simulink model "LDPC_sim"  (R2024a)
(part 11 of 20)

  LDPC Encoder : commblkcod2/LDPC Encoder  ParityCheckMat=sparse([55;2535;8598;9319;10220;14393;26910;27562;145;2625;8688;9409;10310;14483;27000;27652;235;2715;8778;9499;10400;14573;27090;27742;325;2805;8868;9589;10490;14663;27180;27832;415;2895;8958;9679;10580;14753;27270;27922;505;2985;9048;9769;10670;14843;27360;28012;595;3075;9138;9859;10760;14933;27450;28102;685;3165;9228;9949;10850;15023;27540;28192;775;3255;9318;10039;10940;15113;27630;28282;865;3345;9408;10129;11030;15203;27720;28372;955;3435;9498;10219;11120;15293;27810;28462;1045;3525;9588;10309;11210;15383;27900;28552;1135;3615;9678;10399;11300;15473;27990;28642;1225;3705;9768;10489;11390;15563;28080;28732;1315;3795;9858;10579;11480;15653;28170;28822;1405;3885;9948;10669;11570;15743;28260;28912;1495;3975;10038;10759;11660;15833;28350;29002;1585;4065;10128;10849;11750;15923;28440;29092;1675;4155;10218;10939;11840;16013;28530;29182;1765;4245;10308;11029;11930;16103;28620;29272;1855;4335;10398;11119;12020;16193;28710;29362;1945;4425;10488;11209;12110;16283;28800;29452;2035;4515;10578;11299;12200;16373;28890;29542;2125;4605;10668;11389;12290;16463;28980;29632;2215;4695;10758;11479;12380;16553;29070;29722;2305;4785;10848;11569;12470;16643;29160;29812;2395;4875;10938;11659;12560;16733;29250;29902;2485;4965;11028;11749;12650;16823;29340;29992;2575;5055;11118;11839;12740;16913;29430;30082;2665;5145;11208;11929;12830;17003;29520;30172;2755;5235;11298;12019;12920;17093;29610;30262;2845;5325;11388;12109;13010;17183;29700;30352;2935;5415;11478;12199;13100;17273;29790;30442;3025;5505;11568;12289;13190;17363;29880;30532;3115;5595;11658;12379;13280;17453;29970;30622;3205;5685;11748;12469;13370;17543;30060;30712;3295;5775;11838;12559;13460;17633;30150;30802;3385;5865;11928;12649;13550;17723;30240;30892;3475;5955;12018;12739;13640;17813;30330;30982;3565;6045;12108;12829;13730;17903;30420;31072;3655;6135;12198;12919;13820;17993;30510;31162;3745;6225;12288;13009;13910;18083;30600;31252;3835;6315;12378;13099;14000;18173;30690;31342;3925;6405;12468;13189;14090;18263;30780;31432;4015;6495;12558;13279;14180;18353;30870;31522;4105;6585;12648;13369;14270;18443;30960;31612;4195;6675;12738;13459;14360;18533;31050;31702;4285;6765;12828;13549;14450;18623;31140;31792;4375;6855;12918;13639;14540;18713;31230;31882;4465;6945;13008;13729;14630;18803;31320;31972;4555;7035;13098;13819;14720;18893;31410;32062;4645;7125;13188;13909;14810;18983;31500;32152;4735;7215;13278;13999;14900;19073;31590;32242;4825;7305;13368;14089;14990;19163;31680;32332;22;4915;7395;13458;14179;15080;19253;31770;112;5005;7485;13548;14269;15170;19343;31860;202;5095;7575;13638;14359;15260;19433;31950;292;5185;7665;13728;14449;15350;19523;32040;382;5275;7755;13818;14539;15440;19613;32130;472;5365;7845;13908;14629;15530;19703;32220;562;5455;7935;13998;14719;15620;19793;32310;652;5545;8025;14088;14809;15710;19883;32400;90;742;5635;8115;14178;14899;15800;19973;180;832;5725;8205;14268;14989;15890;20063;270;922;5815;8295;14358;15079;15980;20153;360;1012;5905;8385;14448;15169;16070;20243;450;1102;5995;8475;14538;15259;16160;20333;540;1192;6085;8565;14628;15349;16250;20423;630;1282;6175;8655;14718;15439;16340;20513;720;1372;6265;8745;14808;15529;16430;20603;810;1462;6355;8835;14898;15619;16520;20693;900;1552;6445;8925;14988;15709;16610;20783;990;1642;6535;9015;15078;15799;16700;20873;1080;1732;6625;9105;15168;15889;16790;20963;1170;1822;6715;9195;15258;15979;16880;21053;1260;1912;6805;9285;15348;16069;16970;21143;1350;2002;6895;9375;15438;16159;17060;21233;1440;2092;6985;9465;15528;16249;17150;21323;1530;2182;7075;9555;15618;16339;17240;21413;1620;2272;7165;9645;15708;16429;17330;21503;1710;2362;7255;9735;15798;16519;17420;21593;1800;2452;7345;9825;15888;16609;17510;21683;1890;2542;7435;9915;15978;16699;17600;21773;1980;2632;7525;10005;16068;16789;17690;21863;2070;2722;7615;10095;16158;16879;17780;21953;2160;2812;7705;10185;16248;16969;17870;22043;2250;2902;7795;10275;16338;17059;17960;22133;2340;2992;7885;10365;16428;17149;18050;22223;2430;3082;7975;10455;16518;17239;18140;22313;2520;3172;8065;10545 ...(+2551010 chars)true;true;true;true;true;true;true;true;true;true;true;true;true;true;true;true;true;true;true;true;true;true;true;true;true;true;true;true;true;true;true;true;true;true;true;true;true;true;true;true;true;true;true;true;true;true;true;true;true;true;true;true;true;true;true;true;true;true;true;true;true;true;true;true;true;true;true;true;true;true;true;true;true;true;true;true;true;true;true;true;true;true;true;true;true;true;true;true;true;true;true;true;true;true;true;true;true;true;true;true;true;true;true;true;true;true;true;true;true;true;true;true;true;true;true;true;true;true;true;true;true;true;true;true;true;true;true;true;true;true;true;true;true;true;true;true;true;true;true;true;true;true;true;true;true;true;true;true;true;true;true;true;true;true;true;true;true;true;true;true;true;true;true;true;true;true;true;true;true;true;true;true;true;true;true;true;true;true;true;true;true;true;true;true;true;true;true;true;true;true;true;true;true;true;true;true;true;true;true;true;true;true;true;true;true;true;true;true;true;true;true;true;true;true;true;true;true;true;true;true;true;true;true;true;true;true;true;true;true;true;true;true;true;true;true;true;true;true;true;true;true;true;true;true;true;true;true;true;true;true;true;true;true;true;true;true;true;true;true;true;true;true;true;true;true;true;true;true;true;true;true;true;true;true;true;true;true;true;true;true;true;true;true;true;true;true;true;true;true;true;true;true;true;true;true;true;true;true;true;true;true;true;true;true;true;true;true;true;true;true;true;true;true;true;true;true;true;true;true;true;true;true;true;true;true;true;true;true;true;true;true;true;true;true;true;true;true;true;true;true;true;true;true;true;true;true;true;true;true;true;true;true;true;true;true;true;true;true;true;true;true;true;true;true;true;true;true;true;true;true;true;true;true;true;true;true;true;true;true;true;true;true;true;true;true;true;true;true;true;true;true;true;true;true;true;true;true;true;true;true;true;true;true;true;true;true;true;true;true;true;true;true;true;true;true;true;true;true;true;true;true;true;true;true;true;true;true;true;true;true;true;true;true;true;true;true;true;true;true;true;true;true;true;true;true;true;true;true;true;true;true;true;true;true;true;true;true;true;true;true;true;true;true;true;true;true;true;true;true;true;true;true;true;true;true;true;true;true;true;true;true;true;true;true;true;true;true;true;true;true;true;true;true;true;true;true;true;true;true;true;true;true;true;true;true;true;true;true;true;true;true;true;true;true;true;true;true;true;true;true;true;true;true;true;true;true;true;true;true;true;true;true;true;true;true;true;true;true;true;true;true;true;true;true;true;true;true;true;true;true;true;true;true;true;true;true;true;true;true;true;true;true;true;true;true;true;true;true;true;true;true;true;true;true;true;true;true;true;true;true;true;true;true;true;true;true;true;true;true;true;true;true;true;true;true;true;true;true;true;true;true;true;true;true;true;true;true;true;true;true;true;true;true;true;true;true;true;true;true;true;true;true;true;true;true;true;true;true;true;true;true;true;true;true;true;true;true;true;true;true;true;true;true;true;true;true;true;true;true;true;true;true;true;true;true;true;true;true;true;true;true;true;true;true;true;true;true;true;true;true;true;true;true;true;true;true;true;true;true;true;true;true;true;true;true;true;true;true;true;true;true;true;true;true;true;true;true;true;true;true;true;true;true;true;true;true;true;true;true;true;true;true;true;true;true;true;true;true;true;true;true;true;true;true;true;true;true;true;true;true;true;true;true;true;true;true;true;true;true;true;true;true;true;true;true;true;true;true;true;true;true;true;true;true;true;true;true;true;true;true;true;true;true;true;true;true;true;true;true;true;true;true;true;true;true;true;true;true;true;true;true;true;true;true;true;true;true;true;true;true;true;true;true;true;true;true;true;true;true;true;true;true;true;true;true;true;true;true;true;true;true;true;true;true;true;true;true;true;true;true;true;true;true;true;true;true;true;true;true;true;true;true;true;true;true;true;true;true;true;true;true;true;true;true;true;true;true;true;true;true;true;true;true;true;true;true;true;true;true;true;true;true;true;true;true;true;true;true;true;true;true;true;true;true;true;true;true;true;true;true;true;true;true;true;true;true;true;true;true;true;true;true;true;true;true;true;true;true;true;true;true;true;true;true;true;true;true;true;true;true;true;true;true;true;true;true;true;true;true;true;true;true;true;true;true;true;true;true;true;true;true;true;true;true;true;true;true;true;true;true;true;true;true;true;true;true;true;true;true;true;true;true;true;true;true;true;true;true;true;true;true;true;true;true;true;true;true;true;true;true;true;true;true;true;true;true;true;true;true;true;true;true;true;true;true;true;true;true;true;true;true;true;true;true;true;true;true;true;true;true;true;true;true;true;true;true;true;true;true;true;true;true;true;true;true;true;true;true;true;true;true;true;true;true;true;true;true;true;true;true;true;true;true;true;true;true;true;true;true;true;true;true;true;true;true;true;true;true;true;true;true;true;true;true;true;true;true;true;true;true;true;true;true;true;true;true;true;true;true;true;true;true;true;true;true;true;true;true;true;true;true;true;true;true;true;true;true;true;true;true;true;true;true;true;true;true;true;true;true;true;true;true;true;true;true;true;true;true;true;true;true;true;true;true;true;true;true;true;true;true;true;true;true;true;true;true;true;true;true;true;true;true;true;true;true;true;true;true;true;true;true;true;true;true;true;true;true;true;true;true;true;true;true;true;true;true;true;true;true;true;true;true;true;true;true;true;true;true;true;true;true;true;true;true;true;true;true;true;true;true;true;true;true;true;true;true;true;true;true;true;true;true;true;true;true;true;true;true;true;true;true;true;true;true;true;true;true;true;true;true;true;true;true;true;true;true;true;true;true;true;true;true;true;true;true;true;true;true;true;true;true;true;true;true;true;true;true;true;true;true;true;true;true;true;true;true;true;true;true;true;true;true;true;true;true;true;true;true;true;true;true;true;true;true;true;true;true;true;true;true;true;true;true;true;true;true;true;true;true;true;true;true;true;true;true;true;true;true;true;true;true;true;true;true;true;true;true;true;true;true;true;true;true;true;true;true;true;true;true;true;true;true;true;true;true;true;true;true;true;true;true;true;true;true;true;true;true;true;true;true;true;true;true;true;true;true;true;true;true;true;true;true;true;true;true;true;true;true;true;true;true;true;true;true;true;true;true;true;true;true;true;true;true;true;true;true;true;true;true;true;true;true;true;true;true;true;true;true;true;true;true;true;true;true;true;true;true;true;true;true;true;true;true;true;true;true;true;true;true;true;true;true;true;true;true;true;true;true;true;true;true;true;true;true;true;true;true;true;true;true;true;true;true;true;true;true;true;true;true;true;true;true;true;true;true;true;true;true;true;true;true;true;true;true;true;true;true;true;true;true;true;true;true;true;true;true;true;true;true;true;true;true;true;true;true;true;true;true;true;true;true;true;true;true;true;true;true;true;true;true;true;true;true;true;true;true;true;true;true;true;true;true;true;true;true;true;true;true;true;true;true;true;true;true;true;true;true;true;true;true;true;true;true;true;true;true;true;true;true;true;true;true;true;true;true;true;true;true;true;true;true;true;true;true;true;true;true;true;true;true;true;true;true;true;true;true;true;true;true;true;true;true;true;true;true;true;true;true;true;true;true;true;true;true;true;true;true;true;true;true;true;true;true;true;true;true;true;true;true;true;true;true;true;true;true;true;true;true;true;true;true;true;true;true;true;true;true;true;true;true;true;true;true;true;true;true;true;true;true;true;true;true;true;true;true;true;true;true;true;true;true;true;true;true;true;true;true;true;true;true;true;true;true;true;true;true;true;true;true;true;true;true;true;true;true;true;true;true;true;true;true;true;true;true;true;true;true;true;true;true;true;true;true;true;true;true;true;true;true;true;true;true;true;true;true;true;true;true;true;true;true;true;true;true;true;true;true;true;true;true;true;true;true;true;true;true;true;true;true;true;true;true;true;true;true;true;true;true;true;true;true;true;true;true;true;true;true;true;true;true;true;true;true;true;true;true;true;true;true;true;true;true;true;true;true;true;true;true;true;true;true;true;true;true;true;true;true;true;true;true;true;true;true;true;true;true;true;true;true;true;true;true;true;true;true;true;true;true;true;true;true;true;true;true;true;true;true;true;true;true;true;true;true;true;true;true;true;true;true;true;true;true;true;true;true;true;true;true;true;true;true;true;true;true;true;true;true;true;true;true;true;true;true;true;true;true;true;true;true;true;true;true;true;true;true;true;true;true;true;true;true;true;true;true;true;true;true;true;true;true;true;true;true;true;true;true;true;true;true;true;true;true;true;true;true;true;true;true;true;true;true;true;true;true;true;true;true;true;true;true;true;true;true;true;true;true;true;true;true;true;true;true;true;true;true;true;true;true;true;true;true;true;true;true;true;true;true;true;true;true;true;true;true;true;true;true;true;true;true;true;true;true;true;true;true;true;true;true;true;true;true;true;true;true;true;true;true;true;true;true;true;true;true;true;true;true;true;true;true;true;true;true;true;true;true;true;true;true;true;true;true;true;true;true;true;true;true;true;true;true;true;true;true;true;true;true;true;true;true;true;true;true;true;true;true;true;true;true;true;true;true;true;true;true;true;true;true;true;true;true;true;true;true;true;true;true;true;true;true;true;true;true;true;true;true;true;true;true;true;true;true;true;true;true;true;true;true;true;true;true;true;true;true;true;true;true;true;true;true;true;true;true;true;true;true;true;true;true;true;true;true;true;true;true;true;true;true;true;true;true;true;true;true;true;true;true;true;true;true;true;true;true;true;true;true;true;true;true;true;true;true;true;true;true;true;true;true;true;true;true;true;true;true;true;true;true;true;true;true;true;true;true;true;true;true;true;true;true;true;true;true;true;true;true;true;true;true;true;true;true;true;true;true;true;true;true;true;true;true;true;true;true;true;true;true;true;true;true;true;true;true;true;true;true;true;true;true;true;true;true;true;true;true;true;true;true;true;true;true;true;true;true;true;true;true;true;true;true;true;true;true;true;true;true;true;true;true;true;true;true;true;true;true;true;true;true;true;true;true;true;true;true;true;true;true;true;true;true;true;true;true;true;true;true;true;true;true;true;true;true;true;true;true;true;true;true;true;true;true;true;true;true;true;true;true;true;true;true;true;true;true;true;true;true;true;true;true;true;true;true;true;true;true;true;true;true;true;true;true;true;true;true;true;true;true;true;true;true;true;true;true;true;true;true;true;true;true;true;true;true;true;true;true;true;true;true;true;true;true;true;true;true;true;true;true;true;true;true;true;true;true;true;true;true;true;true;true;true;true;true;true;true;true;true;true;true;true;true;true;true;true;true;true;true;true;true;true;true;true;true;true;true;true;true;true;true;true;true;true;true;true;true;true;true;true;true;true;true;true;true;true;true;true;true;true;true;true;true;true;true;true;true;true;true;true;true;true;true;true;true;true;true;true;true;true;true;true;true;true;true;true;true;true;true;true;true;true;true;true;true;true;true;true;true;true;true;true;true;true;true;true;true;true;true;true;true;true;true;true;true;true;true;true;true;true;true;true;true;true;true;true;true;true;true;true;true;true;true;true;true;true;true;true;true;true;true;true;true;true;true;true;true;true;true;true;true;true;true;true;true;true;true;true;true;true;true;true;true;true;true;true;true;true;true;true;true;true;true;true;true;true;true;true;true;true;true;true;true;true;true;true;true;true;true;true;true;true;true;true;true;true;true;true;true;true;true;true;true;true;true;true;true;true;true;true;true;true;true;true;true;true;true;true;true;true;true;true;true;true;true;true;true;true;true;true;true;true;true;true;true;true;true;true;true;true;true;true;true;true;true;true;true;true;true;true;true;true;true;true;true;true;true;true;true;true;true;true;true;true;true;true;true;true;true;true;true;true;true;true;true;true;true;true;true;true;true;true;true;true;true;true;true;true;true;true;true;true;true;true;true;true;true;true;true;true;true;true;true;true;true;true;true;true;true;true;true;true;true;true;true;true;true;true;true;true;true;true;true;true;true;true;true;true;true;true;true;true;true;true;true;true;true;true;true;true;true;true;true;true;true;true;true;true;true;true;true;true;true;true;true;true;true;true;true;true;true;true;true;true;true;true;true;true;true;true;true;true;true;true;true;true;true;true;true;true;true;true;true;true;true;true;true;true;true;true;true;true;true;true;true;true;true;true;true;true;true;true;true;true;true;true;true;true;true;true;true;true;true;true;true;true;true;true;true;true;true;true;true;true;true;true;true;true;true;true;true;true;true;true;true;true;true;true;true;true;true;true;true;true;true;true;true;true;true;true;true;true;true;true;true;true;true;true;true;true;true;true;true;true;true;true;true;true;true;true;true;true;true;true;true;true;true;true;true;true;true;true;true;true;true;true;true;true;true;true;true;true;true;true;true;true;true;true;true;true;true;true;true;true;true;true;true;true;true;true;true;true;true;true;true;true;true;true;true;true;true;true;true;true;true;true;true;true;true;true;true;true;true;true;true;true;true;true;true;true;true;true;true;true;true;true;true;true;true;true;true;true;true;true;true;true;true;true;true;true;true;true;true;true;true;true;true;true;true;true;true;true;true;true;true;true;true;true;true;true;true;true;true;true;true;true;true;true;true;true;true;true;true;true;true;true;true;true;true;true;true;true;true;true;true;true;true;true;true;true;true;true;true;true;true;true;true;true;true;true;true;true;true;true;true;true;true;true;true;true;true;true;true;true;true;true;true;true;true;true;true;true;true;true;true;true;true;true;true;true;true;true;true;true;true;true;true;true;true;true;true;true;true;true;true;true;true;true;true;true;true;true;true;true;true;true;true;true;true;true;true;true;true;true;true;true;true;true;true;true;true;true;true;true;true;true;true;true;true;true;true;true;true;true;true;true;true;true;true;true;true;true;true;true;true;true;true;true;true;true;true;true;true;true;true;true;true;true;true;true;true;true;true;true;true;true;true;true;true;true;true;true;true;true;true;true;true;true;true;true;true;true;true;true;true;true;true;true;true;true;true;true;true;true;true;true;true;true;true;true;true;true;true;true;true;true;true;true;true;true;true;true;true;true;true;true;true;true;true;true;true;true;true;true;true;true;true;true;true;true;true;true;true;true;true;true;true;true;true;true;true;true;true;true;true;true;true;true;true;true;true;true;true;true;true;true;true;true;true;true;true;true;true;true;true;true;true;true;true;true;true;true;true;true;true;true;true;true;true;true;true;true;true;true;true;true;true;true;true;true;true;true;true;true;true;true;true;true;true;true;true;true;true;true;true;true;true;true;true;true;true;true;true;true;true;true;true;true;true;true;true;true;true;true;true;true;true;true;true;true;true;true;true;true;true;true;true;true;true;true;true;true;true;true;true;true;true;true;true;true;true;true;true;true;true;true;true;true;true;true;true;true;true;true;true;true;true;true;true;true;true;true;true;true;true;true;true;true;true;true;true;true;true;true;true;true;true;true;true;true;true;true;true;true;true;true;true;true;true;true;true;true;true;true;true;true;true;true;true;true;true;true;true;true;true;true;true;true;true;true;true;true;true;true;true;true;true;true;true;true;true;true;true;true;true;true;true;true;true;true;true;true;true;true;true;true;true;true;true;true;true;true;true;true;true;true;true;true;true;true;true;true;true;true;true;true;true;true;true;true;true;true;true;true;true;true;true;true;true;true;true;true;true;true;true;true;true;true;true;true;true;true;true;true;true;true;true;true;true;true;true;true;true;true;true;true;true;true;true;true;true;true;true;true;true;true;true;true;true;true;true;true;true;true;true;true;true;true;true;true;true;true;true;true;true;true;true;true;true;true;true;true;true;true;true;true;true;true;true;true;true;true;true;true;true;true;true;true;true;true;true;true;true;true;true;true;true;true;true;true;true;true;true;true;true;true;true;true;true;true;true;true;true;true;true;true;true;true;true;true;true;true;true;true;true;true;true;true;true;true;true;true;true;true;true;true;true;true;true;true;true;true;true;true;true;true;true;true;true;true;true;true;true;true;true;true;true;true;true;true;true;true;true;true;true;true;true;true;true;true;true;true;true;true;true;true;true;true;true;true;true;true;true;true;true;true;true;true;true;true;true;true;true;true;true;true;true;true;true;true;true;true;true;true;true;true;true;true;true;true;true;true;true;true;true;true;true;true;true;true;true;true;true;true;true;true;true;true;true;true;true;true;true;true;true;true;true;true;true;true;true;true;true;true;true;true;true;true;true;true;true;true;true;true;true;true;true;true;true;true;true;true;true;true;true;true;true;true;true;true;true;true;true;true;true;true;true;true;true;true;true;true;true;true;true;true;true;true;true;true;true;true;true;true;true;true;true;true;true;true;true;true;true;true;true;true;true;true;true;true;true;true;true;true;true;true;true;true;true;true;true;true;true;true;true;true;true;true;true;true;true;true;true;true;true;true;true;true;true;true;true;true;true;true;true;true;true;true;true;true;true;true;true;true;true;true;true;true;true;true;true;true;true;true;true;true;true;true;true;true;true;true;true;true;true;true;true;true;true;true;true;true;true;true;true;true;true;true;true;true;true;true;true;true;true;true;true;true;true;true;true;true;true;true;true;true;true;true;true;true;true;true;true;true;true;true;true;true;true;true;true;true;true;true;true;true;true;true;true;true;true;true;true;true;true;true;true;true;true;true;true;true;true;true;true;true;true;true;true;true;true;true;true;true;true;true;true;true;true;true;true;true;true;true;true;true;true;true;true;true;true;true;true;true;true;true;true;true;true;true;true;true;true;true;true;true;true;true;true;true;true;true;true;true;true;true;true;true;true;true;true;true;true;true;true;true;true;true;true;true;true;true;true;true;true;true;true;true;true;true;true;true;true;true;true;true;true;true;true;true;true;true;true;true;true;true;true;true;true;true;true;true;true;true;true;true;true;true;true;true;true;true;true;true;true;true;true;true;true;true;true;true;true;true;true;true;true;true;true;true;true;true;true;true;true;true;true;true;true;true;true;true;true;true;true;true;true;true;true;true;true;true;true;true;true;true;true;true;true;true;true;true;true;true;true;true;true;true;true;true;true;true;true;true;true;true;true;true;true;true;true;true;true;true;true;true;true;true;true;true;true;true;true;true;true;true;true;true;true;true;true;true;true;true;true;true;true;true;true;true;true;true;true;true;true;true;true;true;true;true;true;true;true;true;true;true;true;true;true;true;true;true;true;true;true;true;true;true;true;true;true;true;true;true;true;true;true;true;true;true;true;true;true;true;true;true;true;true;true;true;true;true;true;true;true;true;true;true;true;true;true;true;true;true;true;true;true;true;true;true;true;true;true;true;true;true;true;true;true;true;true;true;true;true;true;true;true;true;true;true;true;true;true;true;true;true;true;true;true;true;true;true;true;true;true;true;true;true;true;true;true;true;true;true;true;true;true;true;true;true;true;true;true;true;true;true;true;true;true;true;true;true;true;true;true;true;true;true;true;true;true;true;true;true;true;true;true;true;true;true;true;true;true;true;true;true;true;true;true;true;true;true;true;true;true;true;true;true;true;true;true;true;true;true;true;true;true;true;true;true;true;true;true;true;true;true;true;true;true;true;true;true;true;true;true;true;true;true;true;true;true;true;true;true;true;true;true;true;true;true;true;true;true;true;true;true;true;true;true;true;true;true;true;true;true;true;true;true;true;true;true;true;true;true;true;true;true;true;true;true;true;true;true;true;true;true;true;true;true;true;true;true;true;true;true;true;true;true;true;true;true;true;true;true;true;true;true;true;true;true;true;true;true;true;true;true;true;true;true;true;true;true;true;true;true;true;true;true;true;true;true;true;true;true;true;true;true;true;true;true;true;true;true;true;true;true;true;true;true;true;true;true;true;true;true;true;true;true;true;true;true;true;true;true;true;true;true;true;true;true;true;true;true;true;true;true;true;true;true;true;true;true;true;true;true;true;true;true;true;true;true;true;true;true;true;true;true;true;true;true;true;true;true;true;true;true;true;true;true;true;true;true;true;true;true;true;true;true;true;true;true;true;true;true;true;true;true;true;true;true;true;true;true;true;true;true;true;true;true;true;true;true;true;true;true;true;true;true;true;true;true;true;true;true;true;true;true;true;true;true;true;true;true;true;true;true;true;true;true;true;true;true;true;true;true;true;true;true;true;true;true;true;true;true;true;true;true;true;true;true;true;true;true;true;true;true;true;true;true;true;true;true;true;true;true;true;true;true;true;true;true;true;true;true;true;true;true;true;true;true;true;true;true;true;true;true;true;true;true;true;true;true;true;true;true;true;true;true;true;true;true;true;true;true;true;true;true;true;true;true;true;true;true;true;true;true;true;true;true;true;true;true;true;true;true;true;true;true;true;true;true;true;true;true;true;true;true;true;true;true;true;true;true;true;true;true;true;true;true;true;true;true;true;true;true;true;true;true;true;true;true;true;true;true;true;true;true;true;true;true;true;true;true;true;true;true;true;true;true;true;true;true;true;true;true;true;true;true;true;true;true;true;true;true;true;true;true;true;true;true;true;true;true;true;true;true;true;true;true;true;true;true;true;true;true;true;true;true;true;true;true;true;true;true;true;true;true;true;true;true;true;true;true;true;true;true;true;true;true;true;true;true;true;true;true;true;true;true;true;true;true;true;true;true;true;true;true;true;true;true;true;true;true;true;true;true;true;true;true;true;true;true;true;true;true;true;true;true;true;true;true;true;true;true;true;true;true;true;true;true;true;true;true;true;true;true;true;true;true;true;true;true;true;true;true;true;true;true;true;true;true;true;true;true;true;true;true;true;true;true;true;true;true;true;true;true;true;true;true;true;true;true;true;true;true;true;true;true;true;true;true;true;true;true;true;true;true;true;true;true;true;true;true;true;true;true;true;true;true;true;true;true;true;true;true;true;true;true;true;true;true;true;true;true;true;true;true;true;true;true;true;true;true;true;true;true;true;true;true;true;true;true;true;true;true;true;true;true;true;true;true;true;true;true;true;true;true;true;true;true;true;true;true;true;true;true;true;true;true;true;true;true;true;true;true;true;true;true;true;true;true;true;true;true;true;true;true;true;true;true;true;true;true;true;true;true;true;true;true;true;true;true;true;true;true;true;true;true;true;true;true;true;true;true;true;true;true;true;true;true;true;true;true;true;true;true;true;true;true;true;true;true;true;true;true;true;true;true;true;true;true;true;true;true;true;true;true;true;true;true;true;true;true;true;true;true;true;true;true;true;true;true;true;true;true;true;true;true;true;true;true;true;true;true;true;true;true;true;true;true;true;true;true;true;true;true;true;true;true;true;true;true;true;true;true;true;true;true;true;true;true;true;true;true;true;true;true;true;true;true;true;true;true;true;true;true;true;true;true;true;true;true;true;true;true;true;true;true;true;true;true;true;true;true;true;true;true;true;true;true;true;true;true;true;true;true;true;true;true;true;true;true;true;true;true;true;true;true;true;true;true;true;true;true;true;true;true;true;true;true;true;true;true;true;true;true;true;true;true;true;true;true;true;true;true;true;true;true;true;true;true;true;true;true;true;true;true;true;true;true;true;true;true;true;true;true;true;true;true;true;true;true;true;true;true;true;true;true;true;true;true;true;true;true;true;true;true;true;true;true;true;true;true;true;true;true;true;true;true;true;true;true;true;true;true;true;true;true;true;true;true;true;true;true;true;true;true;true;true;true;true;true;true;true;true;true;true;true;true;true;true;true;true;true;true;true;true;true;true;true;true;true;true;true;true;true;true;true;true;true;true;true;true;true;true;true;true;true;true;true;true;true;true;true;true;true;true;true;true;true;true;true;true;true;true;true;true;true;true;true;true;true;true;true;true;true;true;true;true;true;true;true;true;true;true;true;true;true;true;true;true;true;true;true;true;true;true;true;true;true;true;true;true;true;true;true;true;true;true;true;true;true;true;true;true;true;true;true;true;true;true;true;true;true;true;true;true;true;true;true;true;true;true;true;true;true;true;true;true;true;true;true;true;true;true;true;true;true;true;true;true;true;true;true;true;true;true;true;true;true;true;true;true;true;true;true;true;true;true;true;true;true;true;true;true;true;true;true;true;true;true;true;true;true;true;true;true;true;true;true;true;true;true;true;true;true;true;true;true;true;true;true;true;true;true;true;true;true;true;true;true;true;true;true;true;true;true;true;true;true;true;true;true;true;true;true;true;true;true;true;true;true;true;true;true;true;true;true;true;true;true;true;true;true;true;true;true;true;true;true;true;true;true;true;true;true;true;true;true;true;true;true;true;true;true;true;true;true;true;true;true;true;true;true;true;true;true;true;true;true;true;true;true;true;true;true;true;true;true;true;true;true;true;true;true;true;true;true;true;true;true;true;true;true;true;true;true;true;true;true;true;true;true;true;true;true;true;true;true;true;true;true;true;true;true;true;true;true;true;true;true;true;true;true;true;true;true;true;true;true;true;true;true;true;true;true;true;true;true;true;true;true;true;true;true;true;true;true;true;true;true;true;true;true;true;true;true;true;true;true;true;true;true;true;true;true;true;true;true;true;true;true;true;true;true;true;true;true;true;true;true;true;true;true;true;true;true;true;true;true;true;true;true;true;true;true;true;true;true;true;true;true;true;true;true;true;true;true;true;true;true;true;true;true;true;true;true;true;true;true;true;true;true;true;true;true;true;true;true;true;true;true;true;true;true;true;true;true;true;true;true;true;true;true;true;true;true;true;true;true;true;true;true;true;true;true;true;true;true;true;true;true;true;true;true;true;true;true;true;true;true;true;true;true;true;true;true;true;true;true;true;true;true;true;true;true;true;true;true;true;true;true;true;true;true;true;true;true;true;true;true;true;true;true;true;true;true;true;true;true;true;true;true;true;true;true;true;true;true;true;true;true;true;true;true;true;true;true;true;true;true;true;true;true;true;true;true;true;true;true;true;true;true;true;true;true;true;true;true;true;true;true;true;true;true;true;true;true;true;true;true;true;true;true;true;true;true;true;true;true;true;true;true;true;true;true;true;true;true;true;true;true;true;true;true;true;true;true;true;true;true;true;true;true;true;true;true;true;true;true;true;true;true;true;true;true;true;true;true;true;true;true;true;true;true;true;true;true;true;true;true;true;true;true;true;true;true;true;true;true;true;true;true;true;true;true;true;true;true;true;true;true;true;true;true;true;true;true;true;true;true;true;true;true;true;true;true;true;true;true;true;true;true;true;true;true;true;true;true;true;true;true;true;true;true;true;true;true;true;true;true;true;true;true;true;true;true;true;true;true;true;true;true;true;true;true;true;true;true;true;true;true;true;true;true;true;true;true;true;true;true;true;true;true;true;true;true;true;true;true;true;true;true;true;true;true;true;true;true;true;true;true;true;true;true;true;true;true;true;true;true;true;true;true;true;true;true;true;true;true;true;true;true;true;true;true;true;true;true;true;true;true;true;true;true;true;true;true;true;true;true;true;true;true;true;true;true;true;true;true;true;true;true;true;true;true;true;true;true;true;true;true;true;true;true;true;true;true;true;true;true;true;true;true;true;true;true;true;true;true;true;true;true;true;true;true;true;true;true;true;true;true;true;true;true;true;true;true;true;true;true;true;true;true;true;true;true;true;true;true;true;true;true;true;true;true;true;true;true;true;true;true;true;true;true;true;true;true;true;true;true;true;true;true;true;true;true;true;true;true;true;true;true;true;true;true;true;true;true;true;true;true;true;true;true;true;true;true;true;true;true;true;true;true;true;true;true;true;true;true;true;true;true;true;true;true;true;true;true;true;true;true;true;true;true;true;true;true;true;true;true;true;true;true;true;true;true;true;true;true;true;true;true;true;true;true;true;true;true;true;true;true;true;true;true;true;true;true;true;true;true;true;true;true;true;true;true;true;true;true;true;true;true;true;true;true;true;true;true;true;true;true;true;true;true;true;true;true;true;true;true;true;true;true;true;true;true;true;true;true;true;true;true;true;true;true;true;true;true;true;true;true;true;true;true;true;true;true;true;true;true;true;true;true;true;true;true;true;true;true;true;true;true;true;true;true;true;true;true;true;true;true;true;true;true;true;true;true;true;true;true;true;true;true;true;true;true;true;true;true;true;true;true;true;true;true;true;true;true;true;true;true;true;true;true;true;true;true;true;true;true;true;true;true;true;true;true;true;true;true;true;true;true;true;true;true;true;true;true;true;true;true;true;true;true;true;true;true;true;true;true;true;true;true;true;true;true;true;true;true;true;true;true;true;true;true;true;true;true;true;true;true;true;true;true;true;true;true;true;true;true;true;true;true;true;true;true;true;true;true;true;true;true;true;true;true;true;true;true;true;true;true;true;true;true;true;true;true;true;true;true;true;true;true;true;true;true;true;true;true;true;true;true;true;true;true;true;true;true;true;true;true;true;true;true;true;true;true;true;true;true;true;true;true;true;true;true;true;true;true;true;true;true;true;true;true;true;true;true;true;true;true;true;true;true;true;true;true;true;true;true;true;true;true;true;true;true;true;true;true;true;true;true;true;true;true;true;true;true;true;true;true;true;true;true;true;true;true;true;true;true;true;true;true;true;true;true;true;true;true;true;true;true;true;true;true;true;true;true;true;true;true;true;true;true;true;true;true;true;true;true;true;true;true;true;true;true;true;true;true;true;true;true;true;true;true;true;true;true;true;true;true;true;true;true;true;true;true;true;true;true;true;true;true;true;true;true;true;true;true;true;true;true;true;true;true;true;true;true;true;true;true;true;true;true;true;true;true;true;true;true;true;true;true;true;true;true;true;true;true;true;true;true;true;true;true;true;true;true;true;true;true;true;true;true;true;true;true;true;true;true;true;true;true;true;true;true;true;true;true;true;true;true;true;true;true;true;true;true;true;true;true;true;true;true;true;true;true;true;true;true;true;true;true;true;true;true;true;true;true;true;true;true;true;true;true;true;true;true;true;true;true;true;true;true;true;true;true;true;true;true;true;true;true;true;true;true;true;true;true;true;true;true;true;true;true;true;true;true;true;true;true;true;true;true;true;true;true;true;true;true;true;true;true;true;true;true;true;true;true;true;true;true;true;true;true;true;true;true;true;true;true;true;true;true;true;true;true;true;true;true;true;true;true;true;true;true;true;true;true;true;true;true;true;true;true;true;true;true;true;true;true;true;true;true;true;true;true;true;true;true;true;true;true;true;true;true;true;true;true;true;true;true;true;true;true;true;true;true;true;true;true;true;true;true;true;true;true;true;true;true;true;true;true;true;true;true;true;true;true;true;true;true;true;true;true;true;true;true;true;true;true;true;true;true;true;true;true;true;true;true;true;true;true;true;true;true;true;true;true;true;true;true;true;true;true;true;true;true;true;true;true;true;true;true;true;true;true;true;true;true;true;true;true;true;true;true;true;true;true;true;true;true;true;true;true;true;true;true;true;true;true;true;true;true;true;true;true;true;true;true;true;true;true;true;true;true;true;true;true;true;true;true;true;true;true;true;true;true;true;true;true;true;true;true;true;true;true;true;true;true;true;true;true;true;true;true;true;true;true;true;true;true;true;true;true;true;true;true;true;true;true;true;true;true;true;true;true;true;true;true;true;true;true;true;true;true;true;true;true;true;true;true;true;true;true;true;true;true;true;true;true;true;true;true;true;true;true;true;true;true;true;true;true;true;true;true;true;true;true;true;true;true;true;true;true;true;true;true;true;true;true;true;true;true;true;true;true;true;true;true;true;true;true;true;true;true;true;true;true;true;true;true;true;true;true;true;true;true;true;true;true;true;true;true;true;true;true;true;true;true;true;true;true;true;true;true;true;true;true;true;true;true;true;true;true;true;true;true;true;true;true;true;true;true;true;true;true;true;true;true;true;true;true;true;true;true;true;true;true;true;true;true;true;true;true;true;true;true;true;true;true;true;true;true;true;true;true;true;true;true;true;true;true;true;true;true;true;true;true;true;true;true;true;true;true;true;true;true;true;true;true;true;true;true;true;true;true;true;true;true;true;true;true;true;true;true;true;true;true;true;true;true;true;true;true;true;true;true;true;true;true;true;true;true;true;true;true;true;true;true;true;true;true;true;true;true;true;true;true;true;true;true;true;true;true;true;true;true;true;true;true;true;true;true;true;true;true;true;true;true;true;true;true;true;true;true;true;true;true;true;true;true;true;true;true;true;true;true;true;true;true;true;true;true;true;true;true;true;true;true;true;true;true;true;true;true;true;true;true;true;true;true;true;true;true;true;true;true;true;true;true;true;true;true;true;true;true;true;true;true;true;true;true;true;true;true;true;true;true;true;true;true;true;true;true;true;true;true;true;true;true;true;true;true;true;true;true;true;true;true;true;true;true;true;true;true;true;true;true;true;true;true;true;true;true;true;true;true;true;true;true;true;true;true;true;true;true;true;true;true;true;true;true;true;true;true;true;true;true;true;true;true;true;true;true;true;true;true;true;true;true;true;true;true;true;true;true;true;true;true;true;true;true;true;true;true;true;true;true;true;true;true;true;true;true;true;true;true;true;true;true;true;true;true;true;true;true;true;true;true;true;true;true;true;true;true;true;true;true;true;true;true;true;true;true;true;true;true;true;true;true;true;true;true;true;true;true;true;true;true;true;true;true;true;true;true;true;true;true;true;true;true;true;true;true;true;true;true;true;true;true;true;true;true;true;true;true;true;true;true;true;true;true;true;true;true;true;true;true;true;true;true;true;true;true;true;true;true;true;true;true;true;true;true;true;true;true;true;true;true;true;true;true;true;true;true;true;true;true;true;true;true;true;true;true;true;true;true;true;true;true;true;true;true;true;true;true;true;true;true;true;true;true;true;true;true;true;true;true;true;true;true;true;true;true;true;true;true;true;true;true;true;true;true;true;true;true;true;true;true;true;true;true;true;true;true;true;true;true;true;true;true;true;true;true;true;true;true;true;true;true;true;true;true;true;true;true;true;true;true;true;true;true;true;true;true;true;true;true;true;true;true;true;true;true;true;true;true;true;true;true;true;true;true;true;true;true;true;true;true;true;true;true;true;true;true;true;true;true;true;true;true;true;true;true;true;true;true;true;true;true;true;true;true;true;true;true;true;true;true;true;true;true;true;true;true;true;true;true;true;true;true;true;true;true;true;true;true;true;true;true;true;true;true;true;true;true;true;true;true;true;true;true;true;true;true;true;true;true;true;true;true;true;true;true;true;true;true;true;true;true;true;true;true;true;true;true;true;true;true;true;true;true;true;true;true;true;true;true;true;true;true;true;true;true;true;true;true;true;true;true;true;true;true;true;true;true;true;true;true;true;true;true;true;true;true;true;true;true;true;true;true;true;true;true;true;true;true;true;true;true;true;true;true;true;true;true;true;true;true;true;true;true;true;true;true;true;true;true;true;true;true;true;true;true;true;true;true;true;true;true;true;true;true;true;true;true;true;true;true;true;true;true;true;true;true;true;true;true;true;true;true;true;true;true;true;true;true;true;true;true;true;true;true;true;true;true;true;true;true;true;true;true;true;true;true;true;true;true;true;true;true;true;true;true;true;true;true;true;true;true;true;true;true;true;true;true;true;true;true;true;true;true;true;true;true;true;true;true;true;true;true;true;true;true;true;true;true;true;true;true;true;true;true;true;true;true;true;true;true;true;true;true;true;true;true;true;true;true;true;true;true;true;true;true;true;true;true;true;true;true;true;true;true;true;true;true;true;true;true;true;true;true;true;true;true;true;true;true;true;true;true;true;true;true;true;true;true;true;true;true;true;true;true;true;true;true;true;true;true;true;true;true;true;true;true;true;true;true;true;true;true;true;true;true;true;true;true;true;true;true;true;true;true;true;true;true;true;true;true;true;true;true;true;true;true;true;true;true;true;true;true;true;true;true;true;true;true;true;true;true;true;true;true;true;true;true;true;true;true;true;true;true;true;true;true;true;true;true;true;true;true;true;true;true;true;true;true;true;true;true;true;true;true;true;true;true;true;true;true;true;true;true;true;true;true;true;true;true;true;true;true;true;true;true;true;true;true;true;true;true;true;true;true;true;true;true;true;true;true;true;true;true;true;true;true;true;true;true;true;true;true;true;true;true;true;true;true;true;true;true;true;true;true;true;true;true;true;true;true;true;true;true;true;true;true;true;true;true;true;true;true;true;true;true;true;true;true;true;true;true;true;true;true;true;true;true;true;true;true;true;true;true;true;true;true;true;true;true;true;true;true;true;true;true;true;true;true;true;true;true;true;true;true;true;true;true;true;true;true;true;true;true;true;true;true;true;true;true;true;true;true;true;true;true;true;true;true;true;true;true;true;true;true;true;true;true;true;true;true;true;true;true;true;true;true;true;true;true;true;true;true;true;true;true;true;true;true;true;true;true;true;true;true;true;true;true;true;true;true;true;true;true;true;true;true;true;true;true;true;true;true;true;true;true;true;true;true;true;true;true;true;true;true;true;true;true;true;true;true;true;true;true;true;true;true;true;true;true;true;true;true;true;true;true;true;true;true;true;true;true;true;true;true;true;true;true;true;true;true;true;true;true;true;true;true;true;true;true;true;true;true;true;true;true;true;true;true;true;true;true;true;true;true;true;true;true;true;true;true;true;true;true;true;true;true;true;true;true;true;true;true;true;true;true;true;true;true;true;true;true;true;true;true;true;true;true;true;true;true;true;true;true;true;true;true;true;true;true;true;true;true;true;true;true;true;true;true;true;true;true;true;true;true;true;true;true;true;true;true;true;true;true;true;true;true;true;true;true;true;true;true;true;true;true;true;true;true;true;true;true;true;true;true;true;true;true;true;true;true;true;true;true;true;true;true;true;true;true;true;true;true;true;true;true;true;true;true;true;true;true;true;true;true;true;true;true;true;true;true;true;true;true;true;true;true;true;true;true;true;true;true;true;true;true;true;true;true;true;true;true;true;true;true;true;true;true;true;true;true;true;true;true;true;true;true;true;true;true;true;true;true;true;true;true;true;true;true;true;true;true;true;true;true;true;true;true;true;true;true;true;true;true;true;true;true;true;true;true;true;true;true;true;true;true;true;true;true;true;true;true;true;true;true;true;true;true;true;true;true;true;true;true;true;true;true;true;true;true;true;true;true;true;true;true;true;true;true;true;true;true;true;true;true;true;true;true;true;true;true;true;true;true;true;true;true;true;true;true;true;true;true;true;true;true;true;true;true;true;true;true;true;true;true;true;true;true;true;true;true;true;true;true;true;true;true;true;true;true;true;true;true;true;true;true;true;true;true;true;true;true;true;true;true;true;true;true;true;true;true;true;true;true;true;true;true;true;true;true;true;true;true;true;true;true;true;true;true;true;true;true;true;true;true;true;true;true;true;true;true;true;true;true;true;true;true;true;true;true;true;true;true;true;true;true;true;true;true;true;true;true;true;true;true;true;true;true;true;true;true;true;true;true;true;true;true;true;true;true;true;true;true;true;true;true;true;true;true;true;true;true;true;true;true;true;true;true;true;true;true;true;true;true;true;true;true;true;true;true;true;true;true;true;true;true;true;true;true;true;true;true;true;true;true;true;true;true;true;true;true;true;true;true;true;true;true;true;true;true;true;true;true;true;true;true;true;true;true;true;true;true;true;true;true;true;true;true;true;true;true;true;true;true;true;true;true;true;true;true;true;true;true;true;true;true;true;true;true;true;true;true;true;true;true;true;true;true;true;true;true;true;true;true;true;true;true;true;true;true;true;true;true;true;true;true;true;true;true;true;true;true;true;true;true;true;true;true;true;true;true;true;true;true;true;true;true;true;true;true;true;true;true;true;true;true;true;true;true;true;true;true;true;true;true;true;true;true;true;true;true;true;true;true;true;true;true;true;true;true;true;true;true;true;true;true;true;true;true;true;true;true;true;true;true;true;true;true;true;true;true;true;true;true;true;true;true;true;true;true;true;true;true;true;true;true;true;true;true;true;true;true;true;true;true;true;true;true;true;true;true;true;true;true;true;true;true;true;true;true;true;true;true;true;true;true;true;true;true;true;true;true;true;true;true;true;true;true;true;true;true;true;true;true;true;true;true;true;true;true;true;true;true;true;true;true;true;true;true;true;true;true;true;true;true;true;true;true;true;true;true;true;true;true;true;true;true;true;true;true;true;true;true;true;true;true;true;true;true;true;true;true;true;true;true;true;true;true;true;true;true;true;true;true;true;true;true;true;true;true;true;true;true;true;true;true;true;true;true;true;true;true;true;true;true;true;true;true;true;true;true;true;true;true;true;true;true;true;true;true;true;true;true;true;true;true;true;true;true;true;true;true;true;true;true;true;true;true;true;true;true;true;true;true;true;true;true;true;true;true;true;true;true;true;true;true;true;true;true;true;true;true;true;true;true;true;true;true;true;true;true;true;true;true;true;true;true;true;true;true;true;true;true;true;true;true;true;true;true;true;true;true;true;true;true;true;true;true;true;true;true;true;true;true;true;true;true;true;true;true;true;true;true;true;true;true;true;true;true;true;true;true;true;true;true;true;true;true;true;true;true;true;true;true;true;true;true;true;true;true;true;true;true;true;true;true;true;true;true;true;true;true;true;true;true;true;true;true;true;true;true;true;true;true;true;true;true;true;true;true;true;true;true;true;true;true;true;true;true;true;true;true;true;true;true;true;true;true;true;true;true;true;true;true;true;true;true;true;true;true;true;true;true;true;true;true;true;true;true;true;true;true;true;true;true;true;true;true;true;true;true;true;true;true;true;true;true;true;true;true;true;true;true;true;true;true;true;true;true;true;true;true;true;true;true;true;true;true;true;true;true;true;true;true;true;true;true;true;true;true;true;true;true;true;true;true;true;true;true;true;true;true;true;true;true;true;true;true;true;true;true;true;true;true;true;true;true;true;true;true;true;true;true;true;true;true;true;true;true;true;true;true;true;true;true;true;true;true;true;true;true;true;true;true;true;true;true;true;true;true;true;true;true;true;true;true;true;true;true;true;true;true;true;true;true;true;true;true;true;true;true;true;true;true;true;true;true;true;true;true;true;true;true;true;true;true;true;true;true;true;true;true;true;true;true;true;true;true;true;true;true;true;true;true;true;true;true;true;true;true;true;true;true;true;true;true;true;true;true;true;true;true;true;true;true;true;true;true;true;true;true;true;true;true;true;true;true;true;true;true;true;true;true;true;true;true;true;true;true;true;true;true;true;true;true;true;true;true;true;true;true;true;true;true;true;true;true;true;true;true;true;true;true;true;true;true;true;true;true;true;true;true;true;true;true;true;true;true;true;true;true;true;true;true;true;true;true;true;true;true;true;true;true;true;true;true;true;true;true;true;true;true;true;true;true;true;true;true;true;true;true;true;true;true;true;true;true;true;true;true;true;true;true;true;true;true;true;true;true;true;true;true;true;true;true;true;true;true;true;true;true;true;true;true;true;true;true;true;true;true;true;true;true;true;true;true;true;true;true;true;true;true;true;true;true;true;true;true;true;true;true;true;true;true;true;true;true;true;true;true;true;true;true;true;true;true;true;true;true;true;true;true;true;true;true;true;true;true;true;true;true;true;true;true;true;true;true;true;true;true;true;true;true;true;true;true;true;true;true;true;true;true;true;true;true;true;true;true;true;true;true;true;true;true;true;true;true;true;true;true;true;true;true;true;true;true;true;true;true;true;true;true;true;true;true;true;true;true;true;true;true;true;true;true;true;true;true;true;true;true;true;true;true;true;true;true;true;true;true;true;true;true;true;true;true;true;true;true;true;true;true;true;true;true;true;true;true;true;true;true;true;true;true;true;true;true;true;true;true;true;true;true;true;true;true;true;true;true;true;true;true;true;true;true;true;true;true;true;true;true;true;true;true;true;true;true;true;true;true;true;true;true;true;true;true;true;true;true;true;true;true;true;true;true;true;true;true;true;true;true;true;true;true;true;true;true;true;true;true;true;true;true;true;true;true;true;true;true;true;true;true;true;true;true;true;true;true;true;true;true;true;true;true;true;true;true;true;true;true;true;true;true;true;true;true;true;true;true;true;true;true;true;true;true;true;true;true;true;true;true;true;true;true;true;true;true;true;true;true;true;true;true;true;true;true;true;true;true;true;true;true;true;true;true;true;true;true;true;true;true;true;true;true;true;true;true;true;true;true;true;true;true;true;true;true;true;true;true;true;true;true;true;true;true;true;true;true;true;true;true;true;true;true;true;true;true;true;true;true;true;true;true;true;true;true;true;true;true;true;true;true;true;true;true;true;true;true;true;true;true;true;true;true;true;true;true;true;true;true;true;true;true;true;true;true;true;true;true;true;true;true;true;true;true;true;true;true;true;true;true;true;true;true;true;true;true;true;true;true;true;true;true;true;true;true;true;true;true;true;true;true;true;true;true;true;true;true;true;true;true;true;true;true;true;true;true;true;true;true;true;true;true;true;true;true;true;true;true;true;true;true;true;true;true;true;true;true;true;true;true;true;true;true;true;true;true;true;true;true;true;true;true;true;true;true;true;true;true;true;true;true;true;true;true;true;true;true;true;true;true;true;true;true;true;true;true;true;true;true;true;true;true;true;true;true;true;true;true;true;true;true;true;true;true;true;true;true;true;true;true;true;true;true;true;true;true;true;true;true;true;true;true;true;true;true;true;true;true;true;true;true;true;true;true;true;true;true;true;true;true;true;true;true;true;true;true;true;true;true;true;true;true;true;true;true;true;true;true;true;true;true;true;true;true;true;true;true;true;true;true;true;true;true;true;true;true;true;true;true;true;true;true;true;true;true;true;true;true;true;true;true;true;true;true;true;true;true;true;true;true;true;true;true;true;true;true;true;true;true;true;true;true;true;true;true;true;true;true;true;true;true;true;true;true;true;true;true;true;true;true;true;true;true;true;true;true;true;true;true;true;true;true;true;true;true;true;true;true;true;true;true;true;true;true;true;true;true;true;true;true;true;true;true;true;true;true;true;true;true;true;true;true;true;true;true;true;true;true;true;true;true;true;true;true;true;true;true;true;true;true;true;true;true;true;true;true;true;true;true;true;true;true;true;true;true;true;true;true;true;true;true;true;true;true;true;true;true;true;true;true;true;true;true;true;true;true;true;true;true;true;true;true;true;true;true;true;true;true;true;true;true;true;true;true;true;true;true;true;true;true;true;true;true;true;true;true;true;true;true;true;true;true;true;true;true;true;true;true;true;true;true;true;true;true;true;true;true;true;true;true;true;true;true;true;true;true;true;true;true;true;true;true;true;true;true;true;true;true;true;true;true;true;true;true;true;true;true;true;true;true;true;true;true;true;true;true;true;true;true;true;true;true;true;true;true;true;true;true;true;true;true;true;true;true;true;true;true;true;true;true;true;true;true;true;true;true;true;true;true;true;true;true;true;true;true;true;true;true;true;true;true;true;true;true;true;true;true;true;true;true;true;true;true;true;true;true;true;true;true;true;true;true;true;true;true;true;true;true;true;true;true;true;true;true;true;true;true;true;true;true;true;true;true;true;true;true;true;true;true;true;true;true;true;true;true;true;true;true;true;true;true;true;true;true;true;true;true;true;true;true;true;true;true;true;true;true;true;true;true;true;true;true;true;true;true;true;true;true;true;true;true;true;true;true;true;true;true;true;true;true;true;true;true;true;true;true;true;true;true;true;true;true;true;true;true;true;true;true;true;true;true;true;true;true;true;true;true;true;true;true;true;true;true;true;true;true;true;true;true;true;true;true;true;true;true;true;true;true;true;true;true;true;true;true;true;true;true;true;true;true;true;true;true;true;true;true;true;true;true;true;true;true;true;true;true;true;true;true;true;true;true;true;true;true;true;true;true;true;true;true;true;true;true;true;true;true;true;true;true;true;true;true;true;true;true;true;true;true;true;true;true;true;true;true;true;true;true;true;true;true;true;true;true;true;true;true;true;true;true;true;true;true;true;true;true;true;true;true;true;true;true;true;true;true;true;true;true;true;true;true;true;true;true;true;true;true;true;true;true;true;true;true;true;true;true;true;true;true;true;true;true;true;true;true;true;true;true;true;true;true;true;true;true;true;true;true;true;true;true;true;true;true;true;true;true;true;true;true;true;true;true;true;true;true;true;true;true;true;true;true;true;true;true;true;true;true;true;true;true;true;true;true;true;true;true;true;true;true;true;true;true;true;true;true;true;true;true;true;true;true;true;true;true;true;true;true;true;true;true;true;true;true;true;true;true;true;true;true;true;true;true;true;true;true;true;true;true;true;true;true;true;true;true;true;true;true;true;true;true;true;true;true;true;true;true;true;true;true;true;true;true;true;true;true;true;true;true;true;true;true;true;true;true;true;true;true;true;true;true;true;true;true;true;true;true;true;true;true;true;true;true;true;true;true;true;true;true;true;true;true;true;true;true;true;true;true;true;true;true;true;true;true;true;true;true;true;true;true;true;true;true;true;true;true;true;true;true;true;true;true;true;true;true;true;true;true;true;true;true;true;true;true;true;true;true;true;true;true;true;true;true;true;true;true;true;true;true;true;true;true;true;true;true;true;true;true;true;true;true;true;true;true;true;true;true;true;true;true;true;true;true;true;true;true;true;true;true;true;true;true;true;true;true;true;true;true;true;true;true;true;true;true;true;true;true;true;true;true;true;true;true;true;true;true;true;true;true;true;true;true;true;true;true;true;true;true;true;true;true;true;true;true;true;true;true;true;true;true;true;true;true;true;true;true;true;true;true;true;true;true;true;true;true;true;true;true;true;true;true;true;true;true;true;true;true;true;true;true;true;true;true;true;true;true;true;true;true;true;true;true;true;true;true;true;true;true;true;true;true;true;true;true;true;true;true;true;true;true;true;true;true;true;true;true;true;true;true;true;true;true;true;true;true;true;true;true;true;true;true;true;true;true;true;true;true;true;true;true;true;true;true;true;true;true;true;true;true;true;true;true;true;true;true;true;true;true;true;true;true;true;true;true;true;true;true;true;true;true;true;true;true;true;true;true;true;true;true;true;true;true;true;true;true;true;true;true;true;true;true;true;true;true;true;true;true;true;true;true;true;true;true;true;true;true;true;true;true;true;true;true;true;true;true;true;true;true;true;true;true;true;true;true;true;true;true;true;true;true;true;true;true;true;true;true;true;true;true;true;true;true;true;true;true;true;true;true;true;true;true;true;true;true;true;true;true;true;true;true;true;true;true;true;true;true;true;true;true;true;true;true;true;true;true;true;true;true;true;true;true;true;true;true;true;true;true;true;true;true;true;true;true;true;true;true;true;true;true;true;true;true;true;true;true;true;true;true;true;true;true;true;true;true;true;true;true;true;true;true;true;true;true;true;true;true;true;true;true;true;true;true;true;true;true;true;true;true;true;true;true;true;true;true;true;true;true;true;true;true;true;true;true;true;true;true;true;true;true;true;true;true;true;true;true;true;true;true;true;true;true;true;true;true;true;true;true;true;true;true;true;true;true;true;true;true;true;true;true;true;true;true;true;true;true;true;true;true;true;true;true;true;true;true;true;true;true;true;true;true;true;true;true;true;true;true;true;true;true;true;true;true;true;true;true;true;true;true;true;true;true;true;true;true;true;true;true;true;true;true;true;true;true;true;true;true;true;true;true;true;true;true;true;true;true;true;true;true;true;true;true;true;true;true;true;true;true;true;true;true;true;true;true;true;true;true;true;true;true;true;true;true;true;true;true;true;true;true;true;true;true;true;true;true;true;true;true;true;true;true;true;true;true;true;true;true;true;true;true;true;true;true;true;true;true;true;true;true;true;true;true;true;true;true;true;true;true;true;true;true;true;true;true;true;true;true;true;true;true;true;true;true;true;true;true;true;true;true;true;true;true;true;true;true;true;true;true;true;true;true;true;true;true;true;true;true;true;true;true;true;true;true;true;true;true;true;true;true;true;true;true;true;true;true;true;true;true;true;true;true;true;true;true;true;true;true;true;true;true;true;true;true;true;true;true;true;true;true;true;true;true;true;true;true;true;true;true;true;true;true;true;true;true;true;true;true;true;true;true;true;true;true;true;true;true;true;true;true;true;true;true;true;true;true;true;true;true;true;true;true;true;true;true;true;true;true;true;true;true;true;true;true;true;true;true;true;true;true;true;true;true;true;true;true;true;true;true;true;true;true;true;true;true;true;true;true;true;true;true;true;true;true;true;true;true;true;true;true;true;true;true;true;true;true;true;true;true;true;true;true;true;true;true;true;true;true;true;true;true;true;true;true;true;true;true;true;true;true;true;true;true;true;true;true;true;true;true;true;true;true;true;true;true;true;true;true;true;true;true;true;true;true;true;true;true;true;true;true;true;true;true;true;true;true;true;true;true;true;true;true;true;true;true;true;true;true;true;true;true;true;true;true;true;true;true;true;true;true;true;true;true;true;true;true;true;true;true;true;true;true;true;true;true;true;true;true;true;true;true;true;true;true;true;true;true;true;true;true;true;true;true;true;true;true;true;true;true;true;true;true;true;true;true;true;true;true;true;true;true;true;true;true;true;true;true;true;true;true;true;true;true;true;true;true;true;true;true;true;true;true;true;true;true;true;true;true;true;true;true;true;true;true;true;true;true;true;true;true;true;true;true;true;true;true;true;true;true;true;true;true;true;true;true;true;true;true;true;true;true;true;true;true;true;true;true;true;true;true;true;true;true;true;true;true;true;true;true;true;true;true;true;true;true;true;true;true;true;true;true;true;true;true;true;true;true;true;true;true;true;true;true;true;true;true;true;true;true;true;true;true;true;true;true;true;true;true;true;true;true;true;true;true;true;true;true;true;true;true;true;true;true;true;true;true;true;true;true;true;true;true;true;true;true;true;true;true;true;true;true;true;true;true;true;true;true;true;true;true;true;true;true;true;true;true;true;true;true;true;true;true;true;true;true;true;true;true;true;true;true;true;true;true;true;true;true;true;true;true;true;true;true;true;true;true;true;true;true;true;true;true;true;true;true;true;true;true;true;true;true;true;true;true;true;true;true;true;true;true;true;true;true;true;true;true;true;true;true;true;true;true;true;true;true;true;true;true;true;true;true;true;true;true;true;true;true;true;true;true;true;true;true;true;true;true;true;true;true;true;true;true;true;true;true;true;true;true;true;true;true;true;true;true;true;true;true;true;true;true;true;true;true;true;true;true;true;true;true;true;true;true;true;true;true;true;true;true;true;true;true;true;true;true;true;true;true;true;true;true;true;true;true;true;true;true;true;true;true;true;true;true;true;true;true;true;true;true;true;true;true;true;true;true;true;true;true;true;true;true;true;true;true;true;true;true;true;true;true;true;true;true;true;true;true;true;true;true;true;true;true;true;true;true;true;true;true;true;true;true;true;true;true;true;true;true;true;true;true;true;true;true;true;true;true;true;true;true;true;true;true;true;true;true;true;true;true;true;true;true;true;true;true;true;true;true;true;true;true;true;true;true;true;true;true;true;true;true;true;true;true;true;true;true;true;true;true;true;true;true;true;true;true;true;true;true;true;true;true;true;true;true;true;true;true;true;true;true;true;true;true;true;true;true;true;true;true;true;true;true;true;true;true;true;true;true;true;true;true;true;true;true;true;true;true;true;true;true;true;true;true;true;true;true;true;true;true;true;true;true;true;true;true;true;true;true;true;true;true;true;true;true;true;true;true;true;true;true;true;true;true;true;true;true;true;true;true;true;true;true;true;true;true;true;true;true;true;true;true;true;true;true;true;true;true;true;true;true;true;true;true;true;true;true;true;true;true;true;true;true;true;true;true;true;true;true;true;true;true;true;true;true;true;true;true;true;true;true;true;true;true;true;true;true;true;true;true;true;true;true;true;true;true;true;true;true;true;true;true;true;true;true;true;true;true;true;true;true;true;true;true;true;true;true;true;true;true;true;true;true;true;true;true;true;true;true;true;true;true;true;true;true;true;true;true;true;true;true;true;true;true;true;true;true;true;true;true;true;true;true;true;true;true;true;true;true;true;true;true;true;true;true;true;true;true;true;true;true;true;true;true;true;true;true;true;true;true;true;true;true;true;true;true;true;true;true;true;true;true;true;true;true;true;true;true;true;true;true;true;true;true;true;true;true;true;true;true;true;true;true;true;true;true;true;true;true;true;true;true;true;true;true;true;true;true;true;true;true;true;true;true;true;true;true;true;true;true;true;true;true;true;true;true;true;true;true;true;true;true;true;true;true;true;true;true;true;true;true;true;true;true;true;true;true;true;true;true;true;true;true;true;true;true;true;true;true;true;true;true;true;true;true;true;true;true;true;true;true;true;true;true;true;true;true;true;true;true;true;true;true;true;true;true;true;true;true;true;true;true;true;true;true;true;true;true;true;true;true;true;true;true;true;true;true;true;true;true;true;true;true;true;true;true;true;true;true;true;true;true;true;true;true;true;true;true;true;true;true;true;true;true;true;true;true;true;true;true;true;true;true;true;true;true;true;true;true;true;true;true;true;true;true;true;true;true;true;true;true;true;true;true;true;true;true;true;true;true;true;true;true;true;true;true;true;true;true;true;true;true;true;true;true;true;true;true;true;true;true;true;true;true;true;true;true;true;true;true;true;true;true;true;true;true;true;true;true;true;true;true;true;true;true;true;true;true;true;true;true;true;true;true;true;true;true;true;true;true;true;true;true;true;true;true;true;true;true;true;true;true;true;true;true;true;true;true;true;true;true;true;true;true;true;true;true;true;true;true;true;true;true;true;true;true;true;true;true;true;true;true;true;true;true;true;true;true;true;true;true;true;true;true;true;true;true;true;true;true;true;true;true;true;true;true;true;true;true;true;true;true;true;true;true;true;true;true;true;true;true;true;true;true;true;true;true;true;true;true;true;true;true;true;true;true;true;true;true;true;true;true;true;true;true;true;true;true;true;true;true;true;true;true;true;true;true;true;true;true;true;true;true;true;true;true;true;true;true;true;true;true;true;true;true;true;true;true;true;true;true;true;true;true;true;true;true;true;true;true;true;true;true;true;true;true;true;true;true;true;true;true;true;true;true;true;true;true;true;true;true;true;true;true;true;true;true;true;true;true;true;true;true;true;true;true;true;true;true;true;true;true;true;true;true;true;true;true;true;true;true;true;true;true;true;true;true;true;true;true;true;true;true;true;true;true;true;true;true;true;true;true;true;true;true;true;true;true;true;true;true;true;true;true;true;true;true;true;true;true;true;true;true;true;true;true;true;true;true;true;true;true;true;true;true;true;true;true;true;true;true;true;true;true;true;true;true;true;true;true;true;true;true;true;true;true;true;true;true;true;true;true;true;true;true;true;true;true;true;true;true;true;true;true;true;true;true;true;true;true;true;true;true;true;true;true;true;true;true;true;true;true;true;true;true;true;true;true;true;true;true;true;true;true;true;true;true;true;true;true;true;true;true;true;true;true;true;true;true;true;true;true;true;true;true;true;true;true;true;true;true;true;true;true;true;true;true;true;true;true;true;true;true;true;true;true;true;true;true;true;true;true;true;true;true;true;true;true;true;true;true;true;true;true;true;true;true;true;true;true;true;true;true;true;true;true;true;true;true;true;true;true;true;true;true;true;true;true;true;true;true;true;true;true;true;true;true;true;true;true;true;true;true;true;true;true;true;true;true;true;true;true;true;true;true;true;true;true;true;true;true;true;true;true;true;true;true;true;true;true;true;true;true;true;true;true;true;true;true;true;true;true;true;true;true;true;true;true;true;true;true;true;true;true;true;true;true;true;true;true;true;true;true;true;true;true;true;true;true;true;true;true;true;true;true;true;true;true;true;true;true;true;true;true;true;true;true;true;true;true;true;true;true;true;true;true;true;true;true;true;true;true;true;true;true;true;true;true;true;true;true;true;true;true;true;true;true;true;true;true;true;true;true;true;true;true;true;true;true;true;true;true;true;true;true;true;true;true;true;true;true;true;true;true;true;true;true;true;true;true;true;true;true;true;true;true;true;true;true;true;true;true;true;true;true;true;true;true;true;true;true;true;true;true;true;true;true;true;true;true;true;true;true;true;true;true;true;true;true;true;true;true;true;true;true;true;true;true;true;true;true;true;true;true;true;true;true;true;true;true;true;true;true;true;true;true;true;true;true;true;true;true;true;true;true;true;true;true;true;true;true;true;true;true;true;true;true;true;true;true;true;true;true;true;true;true;true;true;true;true;true;true;true;true;true;true;true;true;true;true;true;true;true;true;true;true;true;true;true;true;true;true;true;true;true;true;true;true;true;true;true;true;true;true;true;true;true;true;true;true;true;true;true;true;true;true;true;true;true;true;true;true;true;true;true;true;true;true;true;true;true;true;true;true;true;true;true;true;true;true;true;true;true;true;true;true;true;true;true;true;true;true;true;true;true;true;true;true;true;true;true;true;true;true;true;true;true;true;true;true;true;true;true;true;true;true;true;true;true;true;true;true;true;true;true;true;true;true;true;true;true;true;true;true;true;true;true;true;true;true;true;true;true;true;true;true;true;true;true;true;true;true;true;true;true;true;true;true;true;true;true;true;true;true;true;true;true;true;true;true;true;true;true;true;true;true;true;true;true;true;true;true;true;true;true;true;true;true;true;true;true;true;true;true;true;true;true;true;true;true;true;true;true;true;true;true;true;true;true;true;true;true;true;true;true;true;true;true;true;true;true;true;true;true;true;true;true;true;true;true;true;true;true;true;true;true;true;true;true;true;true;true;true;true;true;true;true;true;true;true;true;true;true;true;true;true;true;true;true;true;true;true;true;true;true;true;true;true;true;true;true;true;true;true;true;true;true;true;true;true;true;true;true;true;true;true;true;true;true;true;true;true;true;true;true;true;true;true;true;true;true;true;true;true;true;true;true;true;true;true;true;true;true;true;true;true;true;true;true;true;true;true;true;true;true;true;true;true;true;true;true;true;true;true;true;true;true;true;true;true;true;true;true;true;true;true;true;true;true;true;true;true;true;true;true;true;true;true;true;true;true;true;true;true;true;true;true;true;true;true;true;true;true;true;true;true;true;true;true;true;true;true;true;true;true;true;true;true;true;true;true;true;true;true;true;true;true;true;true;true;true;true;true;true;true;true;true;true;true;true;true;true;true;true;true;true;true;true;true;true;true;true;true;true;true;true;true;true;true;true;true;true;true;true;true;true;true;true;true;true;true;true;true;true;true;true;true;true;true;true;true;true;true;true;true;true;true;true;true;true;true;true;true;true;true;true;true;true;true;true;true;true;true;true;true;true;true;true;true;true;true;true;true;true;true;true;true;true;true;true;true;true;true;true;true;true;true;true;true;true;true;true;true;true;true;true;true;true;true;true;true;true;true;true;true;true;true;true;true;true;true;true;true;true;true;true;true;true;true;true;true;true;true;true;true;true;true;true;true;true;true;true;true;true;true;true;true;true;true;true;true;true;true;true;true;true;true;true;true;true;true;true;true;true;true;true;true;true;true;true;true;true;true;true;true;true;true;true;true;true;true;true;true;true;true;true;true;true;true;true;true;true;true;true;true;true;true;true;true;true;true;true;true;true;true;true;true;true;true;true;true;true;true;true;true;true;true;true;true;true;true;true;true;true;true;true;true;true;true;true;true;true;true;true;true;true;true;true;true;true;true;true;true;true;true;true;true;true;true;true;true;true;true;true;true;true;true;true;true;true;true;true;true;true;true;true;true;true;true;true;true;true;true;true;true;true;true;true;true;true;true;true;true;true;true;true;true;true;true;true;true;true;true;true;true;true;true;true;true;true;true;true;true;true;true;true;true;true;true;true;true;true;true;true;true;true;true;true;true;true;true;true;true;true;true;true;true;true;true;true;true;true;true;true;true;true;true;true;true;true;true;true;true;true;true;true;true;true;true;true;true;true;true;true;true;true;true;true;true;true;true;true;true;true;true;true;true;true;true;true;true;true;true;true;true;true;true;true;true;true;true;true;true;true;true;true;true;true;true;true;true;true;true;true;true;true;true;true;true;true;true;true;true;true;true;true;true;true;true;true;true;true;true;true;true;true;true;true;true;true;true;true;true;true;true;true;true;true;true;true;true;true;true;true;true;true;true;true;true;true;true;true;true;true;true;true;true;true;true;true;true;true;true;true;true;true;true;true;true;true;true;true;true;true;true;true;true;true;true;true;true;true;true;true;true;true;true;true;true;true;true;true;true;true;true;true;true;true;true;true;true;true;true;true;true;true;true;true;true;true;true;true;true;true;true;true;true;true;true;true;true;true;true;true;true;true;true;true;true;true;true;true;true;true;true;true;true;true;true;true;true;true;true;true;true;true;true;true;true;true;true;true;true;true;true;true;true;true;true;true;true;true;true;true;true;true;true;true;true;true;true;true;true;true;true;true;true;true;true;true;true;true;true;true;true;true;true;true;true;true;true;true;true;true;true;true;true;true;true;true;true;true;true;true;true;true;true;true;true;true;true;true;true;true;true;true;true;true;true;true;true;true;true;true;true;true;true;true;true;true;true;true;true;true;true;true;true;true;true;true;true;true;true;true;true;true;true;true;true;true;true;true;true;true;true;true;true;true;true;true;true;true;true;true;true;true;true;true;true;true;true;true;true;true;true;true;true;true;true;true;true;true;true;true;true;true;true;true;true;true;true;true;true;true;true;true;true;true;true;true;true;true;true;true;true;true;true;true;true;true;true;true;true;true;true;true;true;true;true;true;true;true;true;true;true;true;true;true;true;true;true;true;true;true;true;true;true;true;true;true;true;true;true;true;true;true;true;true;true;true;true;true;true;true;true;true;true;true;true;true;true;true;true;true;true;true;true;true;true;true;true;true;true;true;true;true;true;true;true;true;true;true;true;true;true;true;true;true;true;true;true;true;true;true;true;true;true;true;true;true;true;true;true;true;true;true;true;true;true;true;true;true;true;true;true;true;true;true;true;true;true;true;true;true;true;true;true;true;true;true;true;true;true;true;true;true;true;true;true;true;true;true;true;true;true;true;true;true;true;true;true;true;true;true;true;true;true;true;true;true;true;true;true;true;true;true;true;true;true;true;true;true;true;true;true;true;true;true;true;true;true;true;true;true;true;true;true;true;true;true;true;true;true;true;true;true;true;true;true;true;true;true;true;true;true;true;true;true;true;true;true;true;true;true;true;true;true;true;true;true;true;true;true;true;true;true;true;true;true;true;true;true;true;true;true;true;true;true;true;true;true;true;true;true;true;true;true;true;true;true;true;true;true;true;true;true;true;true;true;true;true;true;true;true;true;true;true;true;true;true;true;true;true;true;true;true;true;true;true;true;true;true;true;true;true;true;true;true;true;true;true;true;true;true;true;true;true;true;true;true;true;true;true;true;true;true;true;true;true;true;true;true;true;true;true;true;true;true;true;true;true;true;true;true;true;true;true;true;true;true;true;true;true;true;true;true;true;true;true;true;true;true;true;true;true;true;true;true;true;true;true;true;true;true;true;true;true;true;true;true;true;true;true;true;true;true;true;true;true;true;true;true;true;true;true;true;true;true;true;true;true;true;true;true;true;true;true;true;true;true;true;true;true;true;true;true;true;true;true;true;true;true;true;true;true;true;true;true;true;true;true;true;true;true;true;true;true;true;true;true;true;true;true;true;true;true;true;true;true;true;true;true;true;true;true;true;true;true;true;true;true;true;true;true;true;true;true;true;true;true;true;true;true;true;true;true;true;true;true;true;true;true;true;true;true;true;true;true;true;true;true;true;true;true;true;true;true;true;true;true;true;true;true;true;true;true;true;true;true;true;true;true;true;true;true;true;true;true;true;true;true;true;true;true;true;true;true;true;true;true;true;true;true;true;true;true;true;true;true;true;true;true;true;true;true;true;true;true;true;true;true;true;true;true;true;true;true;true;true;true;true;true;true;true;true;true;true;true;true;true;true;true;true;true;true;true;true;true;true;true;true;true;true;true;true;true;true;true;true;true;true;true;true;true;true;true;true;true;true;true;true;true;true;true;true;true;true;true;true;true;true;true;true;true;true;true;true;true;true;true;true;true;true;true;true;true;true;true;true;true;true;true;true;true;true;true;true;true;true;true;true;true;true;true;true;true;true;true;true;true;true;true;true;true;true;true;true;true;true;true;true;true;true;true;true;true;true;true;true;true;true;true;true;true;true;true;true;true;true;true;true;true;true;true;true;true;true;true;true;true;true;true;true;true;true;true;true;true;true;true;true;true;true;true;true;true;true;true;true;true;true;true;true;true;true;true;true;true;true;true;true;true;true;true;true;true;true;true;true;true;true;true;true;true;true;true;true;true;true;true;true;true;true;true;true;true;true;true;true;true;true;true;true;true;true;true;true;true;true;true;true;true;true;true;true;true;true;true;true;true;true;true;true;true;true;true;true;true;true;true;true;true;true;true;true;true;true;true;true;true;true;true;true;true;true;true;true;true;true;true;true;true;true;true;true;true;true;true;true;true;true;true;true;true;true;true;true;true;true;true;true;true;true;true;true;true;true;true;true;true;true;true;true;true;true;true;true;true;true;true;true;true;true;true;true;true;true;true;true;true;true;true;true;true;true;true;true;true;true;true;true;true;true;true;true;true;true;true;true;true;true;true;true;true;true;true;true;true;true;true;true;true;true;true;true;true;true;true;true;true;true;true;true;true;true;true;true;true;true;true;true;true;true;true;true;true;true;true;true;true;true;true;true;true;true;true;true;true;true;true;true;true;true;true;true;true;true;true;true;true;true;true;true;true;true;true;true;true;true;true;true;true;true;true;true;true;true;true;true;true;true;true;true;true;true;true;true;true;true;true;true;true;true;true;true;true;true;true;true;true;true;true;true;true;true;true;true;true;true;true;true;true;true;true;true;true;true;true;true;true;true;true;true;true;true;true;true;true;true;true;true;true;true;true;true;true;true;true;true;true;true;true;true;true;true;true;true;true;true;true;true;true;true;true;true;true;true;true;true;true;true;true;true;true;true;true;true;true;true;true;true;true;true;true;true;true;true;true;true;true;true;true;true;true;true;true;true;true;true;true;true;true;true;true;true;true;true;true;true;true;true;true;true;true;true;true;true;true;true;true;true;true;true;true;true;true;true;true;true;true;true;true;true;true;true;true;true;true;true;true;true;true;true;true;true;true;true;true;true;true;true;true;true;true;true;true;true;true;true;true;true;true;true;true;true;true;true;true;true;true;true;true;true;true;true;true;true;true;true;true;true;true;true;true;true;true;true;true;true;true;true;true;true;true;true;true;true;true;true;true;true;true;true;true;true;true;true;true;true;true;true;true;true;true;true;true;true;true;true;true;true;true;true;true;true;true;true;true;true;true;true;true;true;true;true;true;true;true;true;true;true;true;true;true;true;true;true;true;true;true;true;true;true;true;true;true;true;true;true;true;true;true;true;true;true;true;true;true;true;true;true;true;true;true;true;true;true;true;true;true;true;true;true;true;true;true;true;true;true;true;true;true;true;true;true;true;true;true;true;true;true;true;true;true;true;true;true;true;true;true;true;true;true;true;true;true;true;true;true;true;true;true;true;true;true;true;true;true;true;true;true;true;true;true;true;true;true;true;true;true;true;true;true;true;true;true;true;true;true;true;true;true;true;true;true;true;true;true;true;true;true;true;true;true;true;true;true;true;true;true;true;true;true;true;true;true;true;true;true;true;true;true;true;true;true;true;true;true;true;true;true;true;true;true;true;true;true;true;true;true;true;true;true;true;true;true;true;true;true;true;true;true;true;true;true;true;true;true;true;true;true;true;true;true;true;true;true;true;true;true;true;true;true;true;true;true;true;true;true;true;true;true;true;true;true;true;true;true;true;true;true;true;true;true;true;true;true;true;true;true;true;true;true;true;true;true;true;true;true;true;true;true;true;true;true;true;true;true;true;true;true;true;true;true;true;true;true;true;true;true;true;true;true;true;true;true;true;true;true;true;true;true;true;true;true;true;true;true;true;true;true;true;true;true;true;true;true;true;true;true;true;true;true;true;true;true;true;true;true;true;true;true;true;true;true;true;true;true;true;true;true;true;true;true;true;true;true;true;true;true;true;true;true;true;true;true;true;true;true;true;true;true;true;true;true;true;true;true;true;true;true;true;true;true;true;true;true;true;true;true;true;true;true;true;true;true;true;true;true;true;true;true;true;true;true;true;true;true;true;true;true;true;true;true;true;true;true;true;true;true;true;true;true;true;true;true;true;true;true;true;true;true;true;true;true;true;true;true;true;true;true;true;true;true;true;true;true;true;true;true;true;true;true;true;true;true;true;true;true;true;true;true;true;true;true;true;true;true;true;true;true;true;true;true;true;true;true;true;true;true;true;true;true;true;true;true;true;true;true;true;true;true;true;true;true;true;true;true;true;true;true;true;true;true;true;true;true;true;true;true;true;true;true;true;true;true;true;true;true;true;true;true;true;true;true;true;true;true;true;true;true;true;true;true;true;true;true;true;true;true;true;true;true;true;true;true;true;true;true;true;true;true;true;true;true;true;true;true;true;true;true;true;true;true;true;true;true;true;true;true;true;true;true;true;true;true;true;true;true;true;true;true;true;true;true;true;true;true;true;true;true;true;true;true;true;true;true;true;true;true;true;true;true;true;true;true;true;true;true;true;true;true;true;true;true;true;true;true;true;true;true;true;true;true;true;true;true;true;true;true;true;true;true;true;true;true;true;true;true;true;true;true;true;true;true;true;true;true;true;true;true;true;true;true;true;true;true;true;true;true;true;true;true;true;true;true;true;true;true;true;true;true;true;true;true;true;true;true;true;true;true;true;true;true;true;true;true;true;true;true;true;true;true;true;true;true;true;true;true;true;true;true;true;true;true;true;true;true;true;true;true;true;true;true;true;true;true;true;true;true;true;true;true;true;true;true;true;true;true;true;true;true;true;true;true;true;true;true;true;true;true;true;true;true;true;true;true;true;true;true;true;true;true;true;true;true;true;true;true;true;true;true;true;true;true;true;true;true;true;true;true;true;true;true;true;true;true;true;true;true;true;true;true;true;true;true;true;true;true;true;true;true;true;true;true;true;true;true;true;true;true;true;true;true;true;true;true;true;true;true;true;true;true;true;true;true;true;true;true;true;true;true;true;true;true;true;true;true;true;true;true;true;true;true;true;true;true;true;true;true;true;true;true;true;true;true;true;true;true;true;true;true;true;true;true;true;true;true;true;true;true;true;true;true;true;true;true;true;true;true;true;true;true;true;true;true;true;true;true;true;true;true;true;true;true;true;true;true;true;true;true;true;true;true;true;true;true;true;true;true;true;true;true;true;true;true;true;true;true;true;true;true;true;true;true;true;true;true;true;true;true;true;true;true;true;true;true;true;true;true;true;true;true;true;true;true;true;true;true;true;true;true;true;true;true;true;true;true;true;true;true;true;true;true;true;true;true;true;true;true;true;true;true;true;true;true;true;true;true;true;true;true;true;true;true;true;true;true;true;true;true;true;true;true;true;true;true;true;true;true;true;true;true;true;true;true;true;true;true;true;true;true;true;true;true;true;true;true;true;true;true;true;true;true;true;true;true;true;true;true;true;true;true;true;true;true;true;true;true;true;true;true;true;true;true;true;true;true;true;true;true;true;true;true;true;true;true;true;true;true;true;true;true;true;true;true;true;true;true;true;true;true;true;true;true;true;true;true;true;true;true;true;true;true;true;true;true;true;true;true;true;true;true;true;true;true;true;true;true;true;true;true;true;true;true;true;true;true;true;true;true;true;true;true;true;true;true;true;true;true;true;true;true;true;true;true;true;true;true;true;true;true;true;true;true;true;true;true;true;true;true;true;true;true;true;true;true;true;true;true;true;true;true;true;true;true;true;true;true;true;true;true;true;true;true;true;true;true;true;true;true;true;true;true;true;true;true;true;true;true;true;true;true;true;true;true;true;true;true;true;true;true;true;true;true;true;true;true;true;true;true;true;true;true;true;true;true;true;true;true;true;true;true;true;true;true;true;true;true;true;true;true;true;true;true;true;true;true;true;true;true;true;true;true;true;true;true;true;true;true;true;true;true;true;true;true;true;true;true;true;true;true;true;true;true;true;true;true;true;true;true;true;true;true;true;true;true;true;true;true;true;true;true;true;true;true;true;true;true;true;true;true;true;true;true;true;true;true;true;true;true;true;true;true;true;true;true;true;true;true;true;true;true;true;true;true;true;true;true;true;true;true;true;true;true;true;true;true;true;true;true;true;true;true;true;true;true;true;true;true;true;true;true;true;true;true;true;true;true;true;true;true;true;true;true;true;true;true;true;true;true;true;true;true;true;true;true;true;true;true;true;true;true;true;true;true;true;true;true;true;true;true;true;true;true;true;true;true;true;true;true;true;true;true;true;true;true;true;true;true;true;true;true;true;true;true;true;true;true;true;true;true;true;true;true;true;true;true;true;true;true;true;true;true;true;true;true;true;true;true;true;true;true;true;true;true;true;true;true;true;true;true;true;true;true;true;true;true;true;true;true;true;true;true;true;true;true;true;true;true;true;true;true;true;true;true;true;true;true;true;true;true;true;true;true;true;true;true;true;true;true;true;true;true;true;true;true;true;true;true;true;true;true;true;true;true;true;true;true;true;true;true;true;true;true;true;true;true;true;true;true;true;true;true;true;true;true;true;true;true;true;true;true;true;true;true;true;true;true;true;true;true;true;true;true;true;true;true;true;true;true;true;true;true;true;true;true;true;true;true;true;true;true;true;true;true;true;true;true;true;true;true;true;true;true;true;true;true;true;true;true;true;true;true;true;true;true;true;true;true;true;true;true;true;true;true;true;true;true;true;true;true;true;true;true;true;true;true;true;true;true;true;true;true;true;true;true;true;true;true;true;true;true;true;true;true;true;true;true;true;true;true;true;true;true;true;true;true;true;true;true;true;true;true;true;true;true;true;true;true;true;true;true;true;true;true;true;true;true;true;true;true;true;true;true;true;true;true;true;true;true;true;true;true;true;true;true;true;true;true;true;true;true;true;true;true;true;true;true;true;true;true;true;true;true;true;true;true;true;true;true;true;true;true;true;true;true;true;true;true;true;true;true;true;true;true;true;true;true;true;true;true;true;true;true;true;true;true;true;true;true;true;true;true;true;true;true;true;true;true;true;true;true;true;true;true;true;true;true;true;true;true;true;true;true;true;true;true;true;true;true;true;true;true;true;true;true;true;true;true;true;true;true;true;true;true;true;true;true;true;true;true;true;true;true;true;true;true;true;true;true;true;true;true;true;true;true;true;true;true;true;true;true;true;true;true;true;true;true;true;true;true;true;true;true;true;true;true;true;true;true;true;true;true;true;true;true;true;true;true;true;true;true;true;true;true;true;true;true;true;true;true;true;true;true;true;true;true;true;true;true;true;true;true;true;true;true;true;true;true;true;true;true;true;true;true;true;true;true;true;true;true;true;true;true;true;true;true;true;true;true;true;true;true;true;true;true;true;true;true;true;true;true;true;true;true;true;true;true;true;true;true;true;true;true;true;true;true;true;true;true;true;true;true;true;true;true;true;true;true;true;true;true;true;true;true;true;true;true;true;true;true;true;true;true;true;true;true;true;true;true;true;true;true;true;true;true;true;true;true;true;true;true;true;true;true;true;true;true;true;true;true;true;true;true;true;true;true;true;true;true;true;true;true;true;true;true;true;true;true;true;true;true;true;true;true;true;true;true;true;true;true;true;true;true;true;true;true;true;true;true;true;true;true;true;true;true;true;true;true;true;true;true;true;true;true;true;true;true;true;true;true;true;true;true;true;true;true;true;true;true;true;true;true;true;true;true;true;true;true;true;true;true;true;true;true;true;true;true;true;true;true;true;true;true;true;true;true;true;true;true;true;true;true;true;true;true;true;true;true;true;true;true;true;true;true;true;true;true;true;true;true;true;true;true;true;true;true;true;true;true;true;true;true;true;true;true;true;true;true;true;true;true;true;true;true;true;true;true;true;true;true;true;true;true;true;true;true;true;true;true;true;true;true;true;true;true;true;true;true;true;true;true;true;true;true;true;true;true;true;true;true;true;true;true;true;true;true;true;true;true;true;true;true;true;true;true;true;true;true;true;true;true;true;true;true;true;true;true;true;true;true;true;true;true;true;true;true;true;true;true;true;true;true;true;true;true;true;true;true;true;true;true;true;true;true;true;true;true;true;true;true;true;true;true;true;true;true;true;true;true;true;true;true;true;true;true;true;true;true;true;true;true;true;true;true;true;true;true;true;true;true;true;true;true;true;true;true;true;true;true;true;true;true;true;true;true;true;true;true;true;true;true;true;true;true;true;true;true;true;true;true;true;true;true;true;true;true;true;true;true;true;true;true;true;true;true;true;true;true;true;true;true;true;true;true;true;true;true;true;true;true;true;true;true;true;true;true;true;true;true;true;true;true;true;true;true;true;true;true;true;true;true;true;true;true;true;true;true;true;true;true;true;true;true;true;true;true;true;true;true;true;true;true;true;true;true;true;true;true;true;true;true;true;true;true;true;true;true;true;true;true;true;true;true;true;true;true;true;true;true;true;true;true;true;true;true;true;true;true;true;true;true;true;true;true;true;true;true;true;true;true;true;true;true;true;true;true;true;true;true;true;true;true;true;true;true;true;true;true;true;true;true;true;true;true;true;true;true;true;true;true;true;true;true;true;true;true;true;true;true;true;true;true;true;true;true;true;true;true;true;true;true;true;true;true;true;true;true;true;true;true;true;true;true;true;true;true;true;true;true;true;true;true;true;true;true;true;true;true;true;true;true;true;true;true;true;true;true;true;true;true;true;true;true;true;true;true;true;true;true;true;true;true;true;true;true;true;true;true;true;true;true;true;true;true;true;true;true;true;true;true;true;true;true;true;true;true;true;true;true;true;true;true;true;true;true;true;true;true;true;true;true;true;true;true;true;true;true;true;true;true;true;true;true;true;true;true;true;true;true;true;true;true;true;true;true;true;true;true;true;true;true;true;true;true;true;true;true;true;true;true;true;true;true;true;true;true;true;true;true;true;true;true;true;true;true;true;true;true;true;true;true;true;true;true;true;true;true;true;true;true;true;true;true;true;true;true;true;true;true;true;true;true;true;true;true;true;true;true;true;true;true;true;true;true;true;true;true;true;true;true;true;true;true;true;true;true;true;true;true;true;true;true;true;true;true;true;true;true;true;true;true;true;true;true;true;true;true;true;true;true;true;true;true;true;true;true;true;true;true;true;true;true;true;true;true;true;true;true;true;true;true;true;true;true;true;true;true;true;true;true;true;true;true;true;true;true;true;true;true;true;true;true;true;true;true;true;true;true;true;true;true;true;true;true;true;true;true;true;true;true;true;true;true;true;true;true;true;true;true;true;true;true;true;true;true;true;true;true;true;true;true;true;true;true;true;true;true;true;true;true;true;true;true;true;true;true;true;true;true;true;true;true;true;true;true;true;true;true;true;true;true;true;true;true;true;true;true;true;true;true;true;true;true;true;true;true;true;true;true;true;true;true;true;true;true;true;true;true;true;true;true;true;true;true;true;true;true;true;true;true;true;true;true;true;true;true;true;true;true;true;true;true;true;true;true;true;true;true;true;true;true;true;true;true;true;true;true;true;true;true;true;true;true;true;true;true;true;true;true;true;true;true;true;true;true;true;true;true;true;true;true;true;true;true;true;true;true;true;true;true;true;true;true;true;true;true;true;true;true;true;true;true;true;true;true;true;true;true;true;true;true;true;true;true;true;true;true;true;true;true;true;true;true;true;true;true;true;true;true;true;true;true;true;true;true;true;true;true;true;true;true;true;true;true;true;true;true;true;true;true;true;true;true;true;true;true;true;true;true;true;true;true;true;true;true;true;true;true;true;true;true;true;true;true;true;true;true;true;true;true;true;true;true;true;true;true;true;true;true;true;true;true;true;true;true;true;true;true;true;true;true;true;true;true;true;true;true;true;true;true;true;true;true;true;true;true;true;true;true;true;true;true;true;true;true;true;true;true;true;true;true;true;true;true;true;true;true;true;true;true;true;true;true;true;true;true;true;true;true;true;true;true;true;true;true;true;true;true;true;true;true;true;true;true;true;true;true;true;true;true;true;true;true;true;true;true;true;true;true;true;true;true;true;true;true;true;true;true;true;true;true;true;true;true;true;true;true;true;true;true;true;true;true;true;true;true;true;true;true;true;true;true;true;true;true;true;true;true;true;true;true;true;true;true;true;true;true;true;true;true;true;true;true;true;true;true;true;true;true;true;true;true;true;true;true;true;true;true;true;true;true;true;true;true;true;true;true;true;true;true;true;true;true;true;true;true;true;true;true;true;true;true;true;true;true;true;true;true;true;true;true;true;true;true;true;true;true;true;true;true;true;true;true;true;true;true;true;true;true;true;true;true;true;true;true;true;true;true;true;true;true;true;true;true;true;true;true;true;true;true;true;true;true;true;true;true;true;true;true;true;true;true;true;true;true;true;true;true;true;true;true;true;true;true;true;true;true;true;true;true;true;true;true;true;true;true;true;true;true;true;true;true;true;true;true;true;true;true;true;true;true;true;true;true;true;true;true;true;true;true;true;true;true;true;true;true;true;true;true;true;true;true;true;true;true;true;true;true;true;true;true;true;true;true;true;true;true;true;true;true;true;true;true;true;true;true;true;true;true;true;true;true;true;true;true;true;true;true;true;true;true;true;true;true;true;true;true;true;true;true;true;true;true;true;true;true;true;true;true;true;true;true;true;true;true;true;true;true;true;true;true;true;true;true;true;true;true;true;true;true;true;true;true;true;true;true;true;true;true;true;true;true;true;true;true;true;true;true;true;true;true;true;true;true;true;true;true;true;true;true;true;true;true;true;true;true;true;true;true;true;true;true;true;true;true;true;true;true;true;true;true;true;true;true;true;true;true;true;true;true;true;true;true;true;true;true;true;true;true;true;true;true;true;true;true;true;true;true;true;true;true;true;true;true;true;true;true;true;true;true;true;true;true;true;true;true;true;true;true;true;true;true;true;true;true;true;true;true;true;true;true;true;true;true;true;true;true;true;true;true;true;true;true;true;true;true;true;true;true;true;true;true;true;true;true;true;true;true;true;true;true;true;true;true;true;true;true;true;true;true;true;true;true;true;true;true;true;true;true;true;true;true;true;true;true;true;true;true;true;true;true;true;true;true;true;true;true;true;true;true;true;true;true;true;true;true;true;true;true;true;true;true;true;true;true;true;true;true;true;true;true;true;true;true;true;true;true;true;true;true;true;true;true;true;true;true;true;true;true;true;true;true;true;true;true;true;true;true;true;true;true;true;true;true;true;true;true;true;true;true;true;true;true;true;true;true;true;true;true;true;true;true;true;true;true;true;true;true;true;true;true;true;true;true;true;true;true;true;true;true;true;true;true;true;true;true;true;true;true;true;true;true;true;true;true;true;true;true;true;true;true;true;true;true;true;true;true;true;true;true;true;true;true;true;true;true;true;true;true;true;true;true;true;true;true;true;true;true;true;true;true;true;true;true;true;true;true;true;true;true;true;true;true;true;true;true;true;true;true;true;true;true;true;true;true;true;true;true;true;true;true;true;true;true;true;true;true;true;true;true;true;true;true;true;true;true;true;true;true;true;true;true;true;true;true;true;true;true;true;true;true;true;true;true;true;true;true;true;true;true;true;true;true;true;true;true;true;true;true;true;true;true;true;true;true;true;true;true;true;true;true;true;true;true;true;true;true;true;true;true;true;true;true;true;true;true;true;true;true;true;true;true;true;true;true;true;true;true;true;true;true;true;true;true;true;true;true;true;true;true;true;true;true;true;true;true;true;true;true;true;true;true;true;true;true;true;true;true;true;true;true;true;true;true;true;true;true;true;true;true;true;true;true;true;true;true;true;true;true;true;true;true;true;true;true;true;true;true;true;true;true;true;true;true;true;true;true;true;true;true;true;true;true;true;true;true;true;true;true;true;true;true;true;true;true;true;true;true;true;true;true;true;true;true;true;true;true;true;true;true;true;true;true;true;true;true;true;true;true;true;true;true;true;true;true;true;true;true;true;true;true;true;true;true;true;true;true;true;true;true;true;true;true;true;true;true;true;true;true;true;true;true;true;true;true;true;true;true;true;true;true;true;true;true;true;true;true;true;true;true;true;true;true;true;true;true;true;true;true;true;true;true;true;true;true;true;true;true;true;true;true;true;true;true;true;true;true;true;true;true;true;true;true;true;true;true;true;true;true;true;true;true;true;true;true;true;true;true;true;true;true;true;true;true;true;true;true;true;true;true;true;true;true;true;true;true;true;true;true;true;true;true;true;true;true;true;true;true;true;true;true;true;true;true;true;true;true;true;true;true;true;true;true;true;true;true;true;true;true;true;true;true;true;true;true;true;true;true;true;true;true;true;true;true;true;true;true;true;true;true;true;true;true;true;true;true;true;true;true;true;true;true;true;true;true;true;true;true;true;true;true;true;true;true;true;true;true;true;true;true;true;true;true;true;true;true;true;true;true;true;true;true;true;true;true;true;true;true;true;true;true;true;true;true;true;true;true;true;true;true;true;true;true;true;true;true;true;true;true;true;true;true;true;true;true;true;true;true;true;true;true;true;true;true;true;true;true;true;true;true;true;true;true;true;true;true;true;true;true;true;true;true;true;true;true;true;true;true;true;true;true;true;true;true;true;true;true;true;true;true;true;true;true;true;true;true;true;true;true;true;true;true;true;true;true;true;true;true;true;true;true;true;true;true;true;true;true;true;true;true;true;true;true;true;true;true;true;true;true;true;true;true;true;true;true;true;true;true;true;true;true;true;true;true;true;true;true;true;true;true;true;true;true;true;true;true;true;true;true;true;true;true;true;true;true;true;true;true;true;true;true;true;true;true;true;true;true;true;true;true;true;true;true;true;true;true;true;true;true;true;true;true;true;true;true;true;true;true;true;true;true;true;true;true;true;true;true;true;true;true;true;true;true;true;true;true;true;true;true;true;true;true;true;true;true;true;true;true;true;true;true;true;true;true;true;true;true;true;true;true;true;true;true;true;true;true;true;true;true;true;true;true;true;true;true;true;true;true;true;true;true;true;true;true;true;true;true;true;true;true;true;true;true;true;true;true;true;true;true;true;true;true;true;true;true;true;true;true;true;true;true;true;true;true;true;true;true;true;true;true;true;true;true;true;true;true;true;true;true;true;true;true;true;true;true;true;true;true;true;true;true;true;true;true;true;true;true;true;true;true;true;true;true;true;true;true;true;true;true;true;true;true;true;true;true;true;true;true;true;true;true;true;true;true;true;true;true;true;true;true;true;true;true;true;true;true;true;true;true;true;true;true;true;true;true;true;true;true;true;true;true;true;true;true;true;true;true;true;true;true;true;true;true;true;true;true;true;true;true;true;true;true;true;true;true;true;true;true;true;true;true;true;true;true;true;true;true;true;true;true;true;true;true;true;true;true;true;true;true;true;true;true;true;true;true;true;true;true;true;true;true;true;true;true;true;true;true;true;true;true;true;true;true;true;true;true;true;true;true;true;true;true;true;true;true;true;true;true;true;true;true;true;true;true;true;true;true;true;true;true;true;true;true;true;true;true;true;true;true;true;true;true;true;true;true;true;true;true;true;true;true;true;true;true;true;true;true;true;true;true;true;true;true;true;true;true;true;true;true;true;true;true;true;true;true;true;true;true;true;true;true;true;true;true;true;true;true;true;true;true;true;true;true;true;true;true;true;true;true;true;true;true;true;true;true;true;true;true;true;true;true;true;true;true;true;true;true;true;true;true;true;true;true;true;true;true;true;true;true;true;true;true;true;true;true;true;true;true;true;true;true;true;true;true;true;true;true;true;true;true;true;true;true;true;true;true;true;true;true;true;true;true;true;true;true;true;true;true;true;true;true;true;true;true;true;true;true;true;true;true;true;true;true;true;true;true;true;true;true;true;true;true;true;true;true;true;true;true;true;true;true;true;true;true;true;true;true;true;true;true;true;true;true;true;true;true;true;true;true;true;true;true;true;true;true;true;true;true;true;true;true;true;true;true;true;true;true;true;true;true;true;true;true;true;true;true;true;true;true;true;true;true;true;true;true;true;true;true;true;true;true;true;true;true;true;true;true;true;true;true;true;true;true;true;true;true;true;true;true;true;true;true;true;true;true;true;true;true;true;true;true;true;true;true;true;true;true;true;true;true;true;true;true;true;true;true;true;true;true;true;true;true;true;true;true;true;true;true;true;true;true;true;true;true;true;true;true;true;true;true;true;true;true;true;true;true;true;true;true;true;true;true;true;true;true;true;true;true;true;true;true;true;true;true;true;true;true;true;true;true;true;true;true;true;true;true;true;true;true;true;true;true;true;true;true;true;true;true;true;true;true;true;true;true;true;true;true;true;true;true;true;true;true;true;true;true;true;true;true;true;true;true;true;true;true;true;true;true;true;true;true;true;true;true;true;true;true;true;true;true;true;true;true;true;true;true;true;true;true;true;true;true;true;true;true;true;true;true;true;true;true;true;true;true;true;true;true;true;true;true;true;true;true;true;true;true;true;true;true;true;true;true;true;true;true;true;true;true;true;true;true;true;true;true;true;true;true;true;true;true;true;true;true;true;true;true;true;true;true;true;true;true;true;true;true;true;true;true;true;true;true;true;true;true;true;true;true;true;true;true;true;true;true;true;true;true;true;true;true;true;true;true;true;true;true;true;true;true;true;true;true;true;true;true;true;true;true;true;true;true;true;true;true;true;true;true;true;true;true;true;true;true;true;true;true;true;true;true;true;true;true;true;true;true;true;true;true;true;true;true;true;true;true;true;true;true;true;true;true;true;true;true;true;true;true;true;true;true;true;true;true;true;true;true;true;true;true;true;true;true;true;true;true;true;true;true;true;true;true;true;true;true;true;true;true;true;true;true;true;true;true;true;true;true;true;true;true;true;true;true;true;true;true;true;true;true;true;true;true;true;true;true;true;true;true;true;true;true;true;true;true;true;true;true;true;true;true;true;true;true;true;true;true;true;true;true;true;true;true;true;true;true;true;true;true;true;true;true;true;true;true;true;true;true;true;true;true;true;true;true;true;true;true;true;true;true;true;true;true;true;true;true;true;true;true;true;true;true;true;true;true;true;true;true;true;true;true;true;true;true;true;true;true;true;true;true;true;true;true;true;true;true;true;true;true;true;true;true;true;true;true;true;true;true;true;true;true;true;true;true;true;true;true;true;true;true;true;true;true;true;true;true;true;true;true;true;true;true;true;true;true;true;true;true;true;true;true;true;true;true;true;true;true;true;true;true;true;true;true;true;true;true;true;true;true;true;true;true;true;true;true;true;true;true;true;true;true;true;true;true;true;true;true;true;true;true;true;true;true;true;true;true;true;true;true;true;true;true;true;true;true;true;true;true;true;true;true;true;true;true;true;true;true;true;true;true;true;true;true;true;true;true;true;true;true;true;true;true;true;true;true;true;true;true;true;true;true;true;true;true;true;true;true;true;true;true;true;true;true;true;true;true;true;true;true;true;true;true;true;true;true;true;true;true;true;true;true;true;true;true;true;true;true;true;true;true;true;true;true;true;true;true;true;true;true;true;true;true;true;true;true;true;true;true;true;true;true;true;true;true;true;true;true;true;true;true;true;true;true;true;true;true;true;true;true;true;true;true;true;true;true;true;true;true;true;true;true;true;true;true;true;true;true;true;true;true;true;true;true;true;true;true;true;true;true;true;true;true;true;true;true;true;true;true;true;true;true;true;true;true;true;true;true;true;true;true;true;true;true;true;true;true;true;true;true;true;true;true;true;true;true;true;true;true;true;true;true;true;true;true;true;true;true;true;true;true;true;true;true;true;true;true;true;true;true;true;true;true;true;true;true;true;true;true;true;true;true;true;true;true;true;true;true;true;true;true;true;true;true;true;true;true;true;true;true;true;true;true;true;true;true;true;true;true;true;true;true;true;true;true;true;true;true;true;true;true;true;true;true;true;true;true;true;true;true;true;true;true;true;true;true;true;true;true;true;true;true;true;true;true;true;true;true;true;true;true;true;true;true;true;true;true;true;true;true;true;true;true;true;true;true;true;true;true;true;true;true;true;true;true;true;true;true;true;true;true;true;true;true;true;true;true;true;true;true;true;true;true;true;true;true;true;true;true;true;true;true;true;true;true;true;true;true;true;true;true;true;true;true;true;true;true;true;true;true;true;true;true;true;true;true;true;true;true;true;true;true;true;true;true;true;true;true;true;true;true;true;true;true;true;true;true;true;true;true;true;true;true;true;true;true;true;true;true;true;true;true;true;true;true;true;true;true;true;true;true;true;true;true;true;true;true;true;true;true;true;true;true;true;true;true;true;true;true;true;true;true;true;true;true;true;true;true;true;true;true;true;true;true;true;true;true;true;true;true;true;true;true;true;true;true;true;true;true;true;true;true;true;true;true;true;true;true;true;true;true;true;true;true;true;true;true;true;true;true;true;true;true;true;true;true;true;true;true;true;true;true;true;true;true;true;true;true;true;true;true;true;true;true;true;true;true;true;true;true;true;true;true;true;true;true;true;true;true;true;true;true;true;true;true;true;true;true;true;true;true;true;true;true;true;true;true;true;true;true;true;true;true;true;true;true;true;true;true;true;true;true;true;true;true;true;true;true;true;true;true;true;true;true;true;true;true;true;true;true;true;true;true;true;true;true;true;true;true;true;true;true;true;true;true;true;true;true;true;true;true;true;true;true;true;true;true;true;true;true;true;true;true;true;true;true;true;true;true;true;true;true;true;true;true;true;true;true;true;true;true;true;true;true;true;true;true;true;true;true;true;true;true;true;true;true;true;true;true;true;true;true;true;true;true;true;true;true;true;true;true;true;true;true;true;true;true;true;true;true;true;true;true;true;true;true;true;true;true;true;true;true;true;true;true;true;true;true;true;true;true;true;true;true;true;true;true;true;true;true;true;true;true;true;true;true;true;true;true;true;true;true;true;true;true;true;true;true;true;true;true;true;true;true;true;true;true;true;true;true;true;true;true;true;true;true;true;true;true;true;true;true;true;true;true;true;true;true;true;true;true;true;true;true;true;true;true;true;true;true;true;true;true;true;true;true;true;true;true;true;true;true;true;true;true;true;true;true;true;true;true;true;true;true;true;true;true;true;true;true;true;true;true;true;true;true;true;true;true;true;true;true;true;true;true;true;true;true;true;true;true;true;true;true;true;true;true;true;true;true;true;true;true;true;true;true;true;true;true;true;true;true;true;true;true;true;true;true;true;true;true;true;true;true;true;true;true;true;true;true;true;true;true;true;true;true;true;true;true;true;true;true;true;true;true;true;true;true;true;true;true;true;true;true;true;true;true;true;true;true;true;true;true;true;true;true;true;true;true;true;true;true;true;true;true;true;true;true;true;true;true;true;true;true;true;true;true;true;true;true;true;true;true;true;true;true;true;true;true;true;true;true;true;true;true;true;true;true;true;true;true;true;true;true;true;true;true;true;true;true;true;true;true;true;true;true;true;true;true;true;true;true;true;true;true;true;true;true;true;true;true;true;true;true;true;true;true;true;true;true;true;true;true;true;true;true;true;true;true;true;true;true;true;true;true;true;true;true;true;true;true;true;true;true;true;true;true;true;true;true;true;true;true;true;true;true;true;true;true;true;true;true;true;true;true;true;true;true;true;true;true;true;true;true;true;true;true;true;true;true;true;true;true;true;true;true;true;true;true;true;true;true;true;true;true;true;true;true;true;true;true;true;true;true;true;true;true;true;true;true;true;true;true;true;true;true;true;true;true;true;true;true;true;true;true;true;true;true;true;true;true;true;true;true;true;true;true;true;true;true;true;true;true;true;true;true;true;true;true;true;true;true;true;true;true;true;true;true;true;true;true;true;true;true;true;true;true;true;true;true;true;true;true;true;true;true;true;true;true;true;true;true;true;true;true;true;true;true;true;true;true;true;true;true;true;true;true;true;true;true;true;true;true;true;true;true;true;true;true;true;true;true;true;true;true;true;true;true;true;true;true;true;true;true;true;true;true;true;true;true;true;true;true;true;true;true;true;true;true;true;true;true;true;true;true;true;true;true;true;true;true;true;true;true;true;true;true;true;true;true;true;true;true;true;true;true;true;true;true;true;true;true;true;true;true;true;true;true;true;true;true;true;true;true;true;true;true;true;true;true;true;true;true;true;true;true;true;true;true;true;true;true;true;true;true;true;true;true;true;true;true;true;true;true;true;true;true;true;true;true;true;true;true;true;true;true;true;true;true;true;true;true;true;true;true;true;true;true;true;true;true;true;true;true;true;true;true;true;true;true;true;true;true;true;true;true;true;true;true;true;true;true;true;true;true;true;true;true;true;true;true;true;true;true;true;true;true;true;true;true;true;true;true;true;true;true;true;true;true;true;true;true;true;true;true;true;true;true;true;true;true;true;true;true;true;true;true;true;true;true;true;true;true;true;true;true;true;true;true;true;true;true;true;true;true;true;true;true;true;true;true;true;true;true;true;true;true;true;true;true;true;true;true;true;true;true;true;true;true;true;true;true;true;true;true;true;true;true;true;true;true;true;true;true;true;true;true;true;true;true;true;true;true;true;true;true;true;true;true;true;true;true;true;true;true;true;true;true;true;true;true;true;true;true;true;true;true;true;true;true;true;true;true;true;true;true;true;true;true;true;true;true;true;true;true;true;true;true;true;true;true;true;true;true;true;true;true;true;true;true;true;true;true;true;true;true;true;true;true;true;true;true;true;true;true;true;true;true;true;true;true;true;true;true;true;true;true;true;true;true;true;true;true;true;true;true;true;true;true;true;true;true;true;true;true;true;true;true;true;true;true;true;true;true;true;true;true;true;true;true;true;true;true;true;true;true;true;true;true;true;true;true;true;true;true;true;true;true;true;true;true;true;true;true;true;true;true;true;true;true;true;true;true;true;true;true;true;true;true;true;true;true;true;true;true;true;true;true;true;true;true;true;true;true;true;true;true;true;true;true;true;true;true;true;true;true;true;true;true;true;true;true;true;true;true;true;true;true;true;true;true;true;true;true;true;true;true;true;true;true;true;true;true;true;true;true;true;true;true;true;true;true;true;true;true;true;true;true;true;true;true;true;true;true;true;true;true;true;true;true;true;true;true;true;true;true;true;true;true;true;true;true;true;true;true;true;true;true;true;true;true;true;true;true;true;true;true;true;true;true;true;true;true;true;true;true;true;true;true;true;true;true;true;true;true;true;true;true;true;true;true;true;true;true;true;true;true;true;true;true;true;true;true;true;true;true;true;true;true;true;true;true;true;true;true;true;true;true;true;true;true;true;true;true;true;true;true;true;true;true;true;true;true;true;true;true;true;true;true;true;true;true;true;true;true;true;true;true;true;true;true;true;true;true;true;true;true;true;true;true;true;true;true;true;true;true;true;true;true;true;true;true;true;true;true;true;true;true;true;true;true;true;true;true;true;true;true;true;true;true;true;true;true;true;true;true;true;true;true;true;true;true;true;true;true;true;true;true;true;true;true;true;true;true;true;true;true;true;true;true;true;true;true;true;true;true;true;true;true;true;true;true;true;true;true;true;true;true;true;true;true;true;true;true;true;true;true;true;true;true;true;true;true;true;true;true;true;true;true;true;true;true;true;true;true;true;true;true;true;true;true;true;true;true;true;true;true;true;true;true;true;true;true;true;true;true;true;true;true;true;true;true;true;true;true;true;true;true;true;true;true;true;true;true;true;true;true;true;true;true;true;true;true;true;true;true;true;true;true;true;true;true;true;true;true;true;true;true;true;true;true;true;true;true;true;true;true;true;true;true;true;true;true;true;true;true;true;true;true;true;true;true;true;true;true;true;true;true;true;true;true;true;true;true;true;true;true;true;true;true;true;true;true;true;true;true;true;true;true;true;true;true;true;true;true;true;true;true;true;true;true;true;true;true;true;true;true;true;true;true;true;true;true;true;true;true;true;true;true;true;true;true;true;true;true;true;true;true;true;true;true;true;true;true;true;true;true;true;true;true;true;true;true;true;true;true;true;true;true;true;true;true;true;true;true;true;true;true;true;true;true;true;true;true;true;true;true;true;true;true;true;true;true;true;true;true;true;true;true;true;true;true;true;true;true;true;true;true;true;true;true;true;true;true;true;true;true;true;true;true;true;true;true;true;true;true;true;true;true;true;true;true;true;true;true;true;true;true;true;true;true;true;true;true;true;true;true;true;true;true;true;true;true;true;true;true;true;true;true;true;true;true;true;true;true;true;true;true;true;true;true;true;true;true;true;true;true;true;true;true;true;true;true;true;true;true;true;true;true;true;true;true;true;true;true;true;true;true;true;true;true;true;true;true;true;true;true;true;true;true;true;true;true;true;true;true;true;true;true;true;true;true;true;true;true;true;true;true;true;true;true;true;true;true;true;true;true;true;true;true;true;true;true;true;true;true;true;true;true;true;true;true;true;true;true;true;true;true;true;true;true;true;true;true;true;true;true;true;true;true;true;true;true;true;true;true;true;true;true;true;true;true;true;true;true;true;true;true;true;true;true;true;true;true;true;true;true;true;true;true;true;true;true;true;true;true;true;true;true;true;true;true;true;true;true;true;true;true;true;true;true;true;true;true;true;true;true;true;true;true;true;true;true;true;true;true;true;true;true;true;true;true;true;true;true;true;true;true;true;true;true;true;true;true;true;true;true;true;true;true;true;true;true;true;true;true;true;true;true;true;true;true;true;true;true;true;true;true;true;true;true;true;true;true;true;true;true;true;true;true;true;true;true;true;true;true;true;true;true;true;true;true;true;true;true;true;true;true;true;true;true;true;true;true;true;true;true;true;true;true;true;true;true;true;true;true;true;true;true;true;true;true;true;true;true;true;true;true;true;true;true;true;true;true;true;true;true;true;true;true;true;true;true;true;true;true;true;true;true;true;true;true;true;true;true;true;true;true;true;true;true;true;true;true;true;true;true;true;true;true;true;true;true;true;true;true;true;true;true;true;true;true;true;true;true;true;true;true;true;true;true;true;true;true;true;true;true;true;true;true;true;true;true;true;true;true;true;true;true;true;true;true;true;true;true;true;true;true;true;true;true;true;true;true;true;true;true;true;true;true;true;true;true;true;true;true;true;true;true;true;true;true;true;true;true;true;true;true;true;true;true;true;true;true;true;true;true;true;true;true;true;true;true;true;true;true;true;true;true;true;true;true;true;true;true;true;true;true;true;true;true;true;true;true;true;true;true;true;true;true;true;true;true;true;true;true;true;true;true;true;true;true;true;true;true;true;true;true;true;true;true;true;true;true;true;true;true;true;true;true;true;true;true;true;true;true;true;true;true;true;true;true;true;true;true;true;true;true;true;true;true;true;true;true;true;true;true;true;true;true;true;true;true;true;true;true;true;true;true;true;true;true;true;true;true;true;true;true;true;true;true;true;true;true;true;true;true;true;true;true;true;true;true;true;true;true;true;true;true;true;true;true;true;true;true;true;true;true;true;true;true;true;true;true;true;true;true;true;true;true;true;true;true;true;true;true;true;true;true;true;true;true;true;true;true;true;true;true;true;true;true;true;true;true;true;true;true;true;true;true;true;true;true;true;true;true;true;true;true;true;true;true;true;true;true;true;true;true;true;true;true;true;true;true;true;true;true;true;true;true;true;true;true;true;true;true;true;true;true;true;true;true;true;true;true;true;true;true;true;true;true;true;true;true;true;true;true;true;true;true;true;true;true;true;true;true;true;true;true;true;true;true;true;true;true;true;true;true;true;true;true;true;true;true;true;true;true;true;true;true;true;true;true;true;true;true;true;true;true;true;true;true;true;true;true;true;true;true;true;true;true;true;true;true;true;true;true;true;true;true;true;true;true;true;true;true;true;true;true;true;true;true;true;true;true;true;true;true;true;true;true;true;true;true;true;true;true;true;true;true;true;true;true;true;true;true;true;true;true;true;true;true;true;true;true;true;true;true;true;true;true;true;true;true;true;true;true;true;true;true;true;true;true;true;true;true;true;true;true;true;true;true;true;true;true;true;true;true;true;true;true;true;true;true;true;true;true;true;true;true;true;true;true;true;true;true;true;true;true;true;true;true;true;true;true;true;true;true;true;true;true;true;true;true;true;true;true;true;true;true;true;true;true;true;true;true;true;true;true;true;true;true;true;true;true;true;true;true;true;true;true;true;true;true;true;true;true;true;true;true;true;true;true;true;true;true;true;true;true;true;true;true;true;true;true;true;true;true;true;true;true;true;true;true;true;true;true;true;true;true;true;true;true;true;true;true;true;true;true;true;true;true;true;true;true;true;true;true;true;true;true;true;true;true;true;true;true;true;true;true;true;true;true;true;true;true;true;true;true;true;true;true;true;true;true;true;true;true;true;true;true;true;true;true;true;true;true;true;true;true;true;true;true;true;true;true;true;true;true;true;true;true;true;true;true;true;true;true;true;true;true;true;true;true;true;true;true;true;true;true;true;true;true;true;true;true;true;true;true;true;true;true;true;true;true;true;true;true;true;true;true;true;true;true;true;true;true;true;true;true;true;true;true;true;true;true;true;true;true;true;true;true;true;true;true;true;true;true;true;true;true;true;true;true;true;true;true;true;true;true;true;true;true;true;true;true;true;true;true;true;true;true;true;true;true;true;true;true;true;true;true;true;true;true;true;true;true;true;true;true;true;true;true;true;true;true;true;true;true;true;true;true;true;true;true;true;true;true;true;true;true;true;true;true;true;true;true;true;true;true;true;true;true;true;true;true;true;true;true;true;true;true;true;true;true;true;true;true;true;true;true;true;true;true;true;true;true;true;true;true;true;true;true;true;true;true;true;true;true;true;true;true;true;true;true;true;true;true;true;true;true;true;true;true;true;true;true;true;true;true;true;true;true;true;true;true;true;true;true;true;true;true;true;true;true;true;true;true;true;true;true;true;true;true;true;true;true;true;true;true;true;true;true;true;true;true;true;true;true;true;true;true;true;true;true;true;true;true;true;true;true;true;true;true;true;true;true;true;true;true;true;true;true;true;true;true;true;true;true;true;true;true;true;true;true;true;true;true;true;true;true;true;true;true;true;true;true;true;true;true;true;true;true;true;true;true;true;true;true;true;true;true;true;true;true;true;true;true;true;true;true;true;true;true;true;true;true;true;true;true;true;true;true;true;true;true;true;true;true;true;true;true;true;true;true;true;true;true;true;true;true;true;true;true;true;true;true;true;true;true;true;true;true;true;true;true;true;true;true;true;true;true;true;true;true;true;true;true;true;true;true;true;true;true;true;true;true;true;true;true;true;true;true;true;true;true;true;true;true;true;true;true;true;true;true;true;true;true;true;true;true;true;true;true;true;true;true;true;true;true;true;true;true;true;true;true;true;true;true;true;true;true;true;true;true;true;true;true;true;true;true;true;true;true;true;true;true;true;true;true;true;true;true;true;true;true;true;true;true;true;true;true;true;true;true;true;true;true;true;true;true;true;true;true;true;true;true;true;true;true;true;true;true;true;true;true;true;true;true;true;true;true;true;true;true;true;true;true;true;true;true;true;true;true;true;true;true;true;true;true;true;true;true;true;true;true;true;true;true;true;true;true;true;true;true;true;true;true;true;true;true;true;true;true;true;true;true;true;true;true;true;true;true;true;true;true;true;true;true;true;true;true;true;true;true;true;true;true;true;true;true;true;true;true;true;true;true;true;true;true;true;true;true;true;true;true;true;true;true;true;true;true;true;true;true;true;true;true;true;true;true;true;true;true;true;true;true;true;true;true;true;true;true;true;true;true;true;true;true;true;true;true;true;true;true;true;true;true;true;true;true;true;true;true;true;true;true;true;true;true;true;true;true;true;true;true;true;true;true;true;true;true;true;true;true;true;true;true;true;true;true;true;true;true;true;true;true;true;true;true;true;true;true;true;true;true;true;true;true;true;true;true;true;true;true;true;true;true;true;true;true;true;true;true;true;true;true;true;true;true;true;true;true;true;true;true;true;true;true;true;true;true;true;true;true;true;true;true;true;true;true;true;true;true;true;true;true;true;true;true;true;true;true;true;true;true;true;true;true;true;true;true;true;true;true;true;true;true;true;true;true;true;true;true;true;true;true;true;true;true;true;true;true;true;true;true;true;true;true;true;true;true;true;true;true;true;true;true;true;true;true;true;true;true;true;true;true;true;true;true;true;true;true;true;true;true;true;true;true;true;true;true;true;true;true;true;true;true;true;true;true;true;true;true;true;true;true;true;true;true;true;true;true;true;true;true;true;true;true;true;true;true;true;true;true;true;true;true;true;true;true;true;true;true;true;true;true;true;true;true;true;true;true;true;true;true;true;true;true;true;true;true;true;true;true;true;true;true;true;true;true;true;true;true;true;true;true;true;true;true;true;true;true;true;true;true;true;true;true;true;true;true;true;true;true;true;true;true;true;true;true;true;true;true;true;true;true;true;true;true;true;true;true;true;true;true;true;true;true;true;true;true;true;true;true;true;true;true;true;true;true;true;true;true;true;true;true;true;true;true;true;true;true;true;true;true;true;true;true;true;true;true;true;true;true;true;true;true;true;true;true;true;true;true;true;true;true;true;true;true;true;true;true;true;true;true;true;true;true;true;true;true;true;true;true;true;true;true;true;true;true;true;true;true;true;true;true;true;true;true;true;true;true;true;true;true;true;true;true;true;true;true;true;true;true;true;true;true;true;true;true;true;true;true;true;true;true;true;true;true;true;true;true;true;true;true;true;true;true;true;true;true;true;true;true;true;true;true;true;true;true;true;true;true;true;true;true;true;true;true;true;true;true;true;true;true;true;true;true;true;true;true;true;true;true;true;true;true;true;true;true;true;true;true;true;true;true;true;true;true;true;true;true;true;true;true;true;true;true;true;true;true;true;true;true;true;true;true;true;true;true;true;true;true;true;true;true;true;true;true;true;true;true;true;true;true;true;true;true;true;true;true;true;true;true;true;true;true;true;true;true;true;true;true;true;true;true;true;true;true;true;true;true;true;true;true;true;true;true;true;true;true;true;true;true;true;true;true;true;true;true;true;true;true;true;true;true;true;true;true;true;true;true;true;true;true;true;true;true;true;true;true;true;true;true;true;true;true;true;true;true;true;true;true;true;true;true;true;true;true;true;true;true;true;true;true;true;true;true;true;true;true;true;true;true;true;true;true;true;true;true;true;true;true;true;true;true;true;true;true;true;true;true;true;true;true;true;true;true;true;true;true;true;true;true;true;true;true;true;true;true;true;true;true;true;true;true;true;true;true;true;true;true;true;true;true;true;true;true;true;true;true;true;true;true;true;true;true;true;true;true;true;true;true;true;true;true;true;true;true;true;true;true;true;true;true;true;true;true;true;true;true;true;true;true;true;true;true;true;true;true;true;true;true;true;true;true;true;true;true;true;true;true;true;true;true;true;true;true;true;true;true;true;true;true;true;true;true;true;true;true;true;true;true;true;true;true;true;true;true;true;true;true;true;true;true;true;true;true;true;true;true;true;true;true;true;true;true;true;true;true;true;true;true;true;true;true;true;true;true;true;true;true;true;true;true;true;true;true;true;true;true;true;true;true;true;true;true;true;true;true;true;true;true;true;true;true;true;true;true;true;true;true;true;true;true;true;true;true;true;true;true;true;true;true;true;true;true;true;true;true;true;true;true;true;true;true;true;true;true;true;true;true;true;true;true;true;true;true;true;true;true;true;true;true;true;true;true;true;true;true;true;true;true;true;true;true;true;true;true;true;true;true;true;true;true;true;true;true;true;true;true;true;true;true;true;true;true;true;true;true;true;true;true;true;true;true;true;true;true;true;true;true;true;true;true;true;true;true;true;true;true;true;true;true;true;true;true;true;true;true;true;true;true;true;true;true;true;true;true;true;true;true;true;true;true;true;true;true;true;true;true;true;true;true;true;true;true;true;true;true;true;true;true;true;true;true;true;true;true;true;true;true;true;true;true;true;true;true;true;true;true;true;true;true;true;true;true;true;true;true;true;true;true;true;true;true;true;true;true;true;true;true;true;true;true;true;true;true;true;true;true;true;true;true;true;true;true;true;true;true;true;true;true;true;true;true;true;true;true;true;true;true;true;true;true;true;true;true;true;true;true;true;true;true;true;true;true;true;true;true;true;true;true;true;true;true;true;true;true;true;true;true;true;true;true;true;true;true;true;true;true;true;true;true;true;true;true;true;true;true;true;true;true;true;true;true;true;true;true;true;true;true;true;true;true;true;true;true;true;true;true;true;true;true;true;true;true;true;true;true;true;true;true;true;true;true;true;true;true;true;true;true;true;true;true;true;true;true;true;true;true;true;true;true;true;true;true;true;true;true;true;true;true;true;true;true;true;true;true;true;true;true;true;true;true;true;true;true;true;true;true;true;true;true;true;true;true;true;true;true;true;true;true;true;true;true;true;true;true;true;true;true;true;true;true;true;true;true;true;true;true;true;true;true;true;true;true;true;true;true;true;true;true;true;true;true;true;true;true;true;true;true;true;true;true;true;true;true;true;true;true;true;true;true;true;true;true;true;true;true;true;true;true;true;true;true;true;true;true;true;true;true;true;true;true;true;true;true;true;true;true;true;true;true;true;true;true;true;true;true;true;true;true;true;true;true;true;true;true;true;true;true;true;true;true;true;true;true;true;true;true;true;true;true;true;true;true;true;true;true;true;true;true;true;true;true;true;true;true;true;true;true;true;true;true;true;true;true;true;true;true;true;true;true;true;true;true;true;true;true;true;true;true;true;true;true;true;true;true;true;true;true;true;true;true;true;true;true;true;true;true;true;true;true;true;true;true;true;true;true;true;true;true;true;true;true;true;true;true;true;true;true;true;true;true;true;true;true;true;true;true;true;true;true;true;true;true;true;true;true;true;true;true;true;true;true;true;true;true;true;true;true;true;true;true;true;true;true;true;true;true;true;true;true;true;true;true;true;true;true;true;true;true;true;true;true;true;true;true;true;true;true;true;true;true;true;true;true;true;true;true;true;true;true;true;true;true;true;true;true;true;true;true;true;true;true;true;true;true;true;true;true;true;true;true;true;true;true;true;true;true;true;true;true;true;true;true;true;true;true;true;true;true;true;true;true;true;true;true;true;true;true;true;true;true;true;true;true;true;true;true;true;true;true;true;true;true;true;true;true;true;true;true;true;true;true;true;true;true;true;true;true;true;true;true;true;true;true;true;true;true;true;true;true;true;true;true;true;true;true;true;true;true;true;true;true;true;true;true;true;true;true;true;true;true;true;true;true;true;true;true;true;true;true;true;true;true;true;true;true;true;true;true;true;true;true;true;true;true;true;true;true;true;true;true;true;true;true;true;true;true;true;true;true;true;true;true;true;true;true;true;true;true;true;true;true;true;true;true;true;true;true;true;true;true;true;true;true;true;true;true;true;true;true;true;true;true;true;true;true;true;true;true;true;true;true;true;true;true;true;true;true;true;true;true;true;true;true;true;true;true;true;true;true;true;true;true;true;true;true;true;true;true;true;true;true;true;true;true;true;true;true;true;true;true;true;true;true;true;true;true;true;true;true;true;true;true;true;true;true;true;true;true;true;true;true;true;true;true;true;true;true;true;true;true;true;true;true;true;true;true;true;true;true;true;true;true;true;true;true;true;true;true;true;true;true;true;true;true;true;true;true;true;true;true;true;true;true;true;true;true;true;true;true;true;true;true;true;true;true;true;true;true;true;true;true;true;true;true;true;true;true;true;true;true;true;true;true;true;true;true;true;true;true;true;true;true;true;true;true;true;true;true;true;true;true;true;true;true;true;true;true;true;true;true;true;true;true;true;true;true;true;true;true;true;true;true;true;true;true;true;true;true;true;true;true;true;true;true;true;true;true;true;true;true;true;true;true;true;true;true;true;true;true;true;true;true;true;true;true;true;true;true;true;true;true;true;true;true;true;true;true;true;true;true;true;true;true;true;true;true;true;true;true;true;true;true;true;true;true;true;true;true;true;true;true;true;true;true;true;true;true;true;true;true;true;true;true;true;true;true;true;true;true;true;true;true;true;true;true;true;true;true;true;true;true;true;true;true;true;true;true;true;true;true;true;true;true;true;true;true;true;true;true;true;true;true;true;true;true;true;true;true;true;true;true;true;true;true;true;true;true;true;true;true;true;true;true;true;true;true;true;true;true;true;true;true;true;true;true;true;true;true;true;true;true;true;true;true;true;true;true;true;true;true;true;true;true;true;true;true;true;true;true;true;true;true;true;true;true;true;true;true;true;true;true;true;true;true;true;true;true;true;true;true;true;true;true;true;true;true;true;true;true;true;true;true;true;true;true;true;true;true;true;true;true;true;true;true;true;true;true;true;true;true;true;true;true;true;true;true;true;true;true;true;true;true;true;true;true;true;true;true;true;true;true;true;true;true;true;true;true;true;true;true;true;true;true;true;true;true;true;true;true;true;true;true;true;true;true;true;true;true;true;true;true;true;true;true;true;true;true;true;true;true;true;true;true;true;true;true;true;true;true;true;true;true;true;true;true;true;true;true;true;true;true;true;true;true;true;true;true;true;true;true;true;true;true;true;true;true;true;true;true;true;true;true;true;true;true;true;true;true;true;true;true;true;true;true;true;true;true;true;true;true;true;true;true;true;true;true;true;true;true;true;true;true;true;true;true;true;true;true;true;true;true;true;true;true;true;true;true;true;true;true;true;true;true;true;true;true;true;true;true;true;true;true;true;true;true;true;true;true;true;true;true;true;true;true;true;true;true;true;true;true;true;true;true;true;true;true;true;true;true;true;true;true;true;true;true;true;true;true;true;true;true;true;true;true;true;true;true;true;true;true;true;true;true;true;true;true;true;true;true;true;true;true;true;true;true;true;true;true;true;true;true;true;true;true;true;true;true;true;true;true;true;true;true;true;true;true;true;true;true;true;true;true;true;true;true;true;true;true;true;true;true;true;true;true;true;true;true;true;true;true;true;true;true;true;true;true;true;true;true;true;true;true;true;true;true;true;true;true;true;true;true;true;true;true;true;true;true;true;true;true;true;true;true;true;true;true;true;true;true;true;true;true;true;true;true;true;true;true;true;true;true;true;true;true;true;true;true;true;true;true;true;true;true;true;true;true;true;true;true;true;true;true;true;true;true;true;true;true;true;true;true;true;true;true;true;true;true;true;true;true;true;true;true;true;true;true;true;true;true;true;true;true;true;true;true;true;true;true;true;true;true;true;true;true;true;true;true;true;true;true;true;true;true;true;true;true;true;true;true;true;true;true;true;true;true;true;true;true;true;true;true;true;true;true;true;true;true;true;true;true;true;true;true;true;true;true;true;true;true;true;true;true;true;true;true;true;true;true;true;true;true;true;true;true;true;true;true;true;true;true;true;true;true;true;true;true;true;true;true;true;true;true;true;true;true;true;true;true;true;true;true;true;true;true;true;true;true;true;true;true;true;true;true;true;true;true;true;true;true;true;true;true;true;true;true;true;true;true;true;true;true;true;true;true;true;true;true;true;true;true;true;true;true;true;true;true;true;true;true;true;true;true;true;true;true;true;true;true;true;true;true;true;true;true;true;true;true;true;true;true;true;true;true;true;true;true;true;true;true;true;true;true;true;true;true;true;true;true;true;true;true;true;true;true;true;true;true;true;true;true;true;true;true;true;true;true;true;true;true;true;true;true;true;true;true;true;true;true;true;true;true;true;true;true;true;true;true;true;true;true;true;true;true;true;true;true;true;true;true;true;true;true;true;true;true;true;true;true;true;true;true;true;true;true;true;true;true;true;true;true;true;true;true;true;true;true;true;true;true;true;true;true;true;true;true;true;true;true;true;true;true;true;true;true;true;true;true;true;true;true;true;true;true;true;true;true;true;true;true;true;true;true;true;true;true;true;true;true;true;true;true;true;true;true;true;true;true;true;true;true;true;true;true;true;true;true;true;true;true;true;true;true;true;true;true;true;true;true;true;true;true;true;true;true;true;true;true;true;true;true;true;true;true;true;true;true;true;true;true;true;true;true;true;true;true;true;true;true;true;true;true;true;true;true;true;true;true;true;true;true;true;true;true;true;true;true;true;true;true;true;true;true;true;true;true;true;true;true;true;true;true;true;